simulink model "main"  (R2022a)
settings: Solver=FixedStepDiscrete  StartTime=0.0  StopTime=Inf  FixedStep=(50e-6)-(sim_en*4.995e-5)  RelTol=1e-3  EnableMultiTasking=on
model workspace (MAT data in the model file):
  Param = Simulink.Parameter
  Param.DataType = 'auto'
  Param.Complexity = 'real'
  Param.Dimensions = [0 0]
  ac_ok = Simulink.Signal
  ac_ok.DataType = 'boolean'
  ac_ok.Dimensions = -1
  ac_ok.DimensionsMode = 'Fixed'
  ac_ok.Complexity = 'real'
  ac_ok.SampleTime = -1
  ac_ok.SamplingMode = 'auto'
  ac_ok.InitialValue = '0'
  ac_ok_120 = Simulink.Signal
  ac_ok_120.DataType = 'boolean'
  ac_ok_120.Dimensions = -1
  ac_ok_120.DimensionsMode = 'Fixed'
  ac_ok_120.Complexity = 'real'
  ac_ok_120.SampleTime = -1
  ac_ok_120.SamplingMode = 'auto'
  ac_ok_120.InitialValue = '0'
  bulk_voltage = Simulink.Signal
  bulk_voltage.DataType = 'uint16'
  bulk_voltage.Dimensions = -1
  bulk_voltage.DimensionsMode = 'Fixed'
  bulk_voltage.Complexity = 'real'
  bulk_voltage.SampleTime = -1
  bulk_voltage.SamplingMode = 'auto'
  bulk_voltage.InitialValue = '99'
  burstduty_integ_max = Simulink.Signal
  burstduty_integ_max.DataType = 'single'
  burstduty_integ_max.Dimensions = -1
  burstduty_integ_max.DimensionsMode = 'Fixed'
  burstduty_integ_max.Complexity = 'real'
  burstduty_integ_max.SampleTime = -1
  burstduty_integ_max.SamplingMode = 'auto'
  burstduty_integ_max.InitialValue = '1'
  burstduty_integ_min = Simulink.Signal
  burstduty_integ_min.DataType = 'single'
  burstduty_integ_min.Dimensions = -1
  burstduty_integ_min.DimensionsMode = 'Fixed'
  burstduty_integ_min.Complexity = 'real'
  burstduty_integ_min.SampleTime = -1
  burstduty_integ_min.SamplingMode = 'auto'
  burstduty_integ_min.InitialValue = '1'
  burstduty_ki = Simulink.Signal
  burstduty_ki.DataType = 'single'
  burstduty_ki.Dimensions = -1
  burstduty_ki.DimensionsMode = 'Fixed'
  burstduty_ki.Complexity = 'real'
  burstduty_ki.SampleTime = -1
  burstduty_ki.SamplingMode = 'auto'
  burstduty_ki.InitialValue = '-1'
  burstduty_kp = Simulink.Signal
  burstduty_kp.DataType = 'single'
  burstduty_kp.Dimensions = -1
  burstduty_kp.DimensionsMode = 'Fixed'
  burstduty_kp.Complexity = 'real'
  burstduty_kp.SampleTime = -1
  burstduty_kp.SamplingMode = 'auto'
  burstduty_kp.InitialValue = '-1'
  calib_ok = Simulink.Signal
  calib_ok.DataType = 'boolean'
  calib_ok.Dimensions = -1
  calib_ok.DimensionsMode = 'Fixed'
  calib_ok.Complexity = 'real'
  calib_ok.SampleTime = -1
  calib_ok.SamplingMode = 'auto'
  calib_ok.InitialValue = '0'
  can_addr1 = Simulink.Signal
  can_addr1.DataType = 'boolean'
  can_addr1.Dimensions = -1
  can_addr1.DimensionsMode = 'Fixed'
  can_addr1.Complexity = 'real'
  can_addr1.SampleTime = -1
  can_addr1.SamplingMode = 'auto'
  can_addr1.InitialValue = '0'
  can_addr2 = Simulink.Signal
  can_addr2.DataType = 'boolean'
  can_addr2.Dimensions = -1
  can_addr2.DimensionsMode = 'Fixed'
  can_addr2.Complexity = 'real'
  can_addr2.SampleTime = -1
  can_addr2.SamplingMode = 'auto'
  can_addr2.InitialValue = '0'
  can_addr3 = Simulink.Signal
  can_addr3.DataType = 'boolean'
  can_addr3.Dimensions = -1
  can_addr3.DimensionsMode = 'Fixed'
  can_addr3.Complexity = 'real'
  can_addr3.SampleTime = -1
  can_addr3.SamplingMode = 'auto'
  can_addr3.InitialValue = '0'
  can_addr4 = Simulink.Signal
  can_addr4.DataType = 'boolean'
  can_addr4.Dimensions = -1
  can_addr4.DimensionsMode = 'Fixed'
  can_addr4.Complexity = 'real'
  can_addr4.SampleTime = -1
  can_addr4.SamplingMode = 'auto'
  can_addr4.InitialValue = '0'
  can_data_rx = Simulink.Signal
  can_data_rx.DataType = 'uint8'
  can_data_rx.Dimensions = [1 8]
  can_data_rx.DimensionsMode = 'Fixed'
  can_data_rx.Complexity = 'real'
  can_data_rx.SampleTime = -1
  can_data_rx.SamplingMode = 'auto'
  can_data_rx.InitialValue = '[0 0 0 0 0 0 0 0]'
  can_data_tx = Simulink.Signal
  can_data_tx.DataType = 'uint8'
  can_data_tx.Dimensions = [1 8]
  can_data_tx.DimensionsMode = 'Fixed'
  can_data_tx.Complexity = 'real'
  can_data_tx.SampleTime = -1
  can_data_tx.SamplingMode = 'auto'
  can_data_tx.InitialValue = '[0 0 0 0 0 0 0 0]'
  can_timeout_120 = Simulink.Signal
  can_timeout_120.DataType = 'boolean'
  can_timeout_120.Dimensions = -1
  can_timeout_120.DimensionsMode = 'Fixed'
  can_timeout_120.Complexity = 'real'
  can_timeout_120.SampleTime = -1
  can_timeout_120.SamplingMode = 'auto'
  can_timeout_120.InitialValue = '0'
  chksum_scircv = Simulink.Signal
  chksum_scircv.DataType = 'boolean'
  chksum_scircv.Dimensions = -1
  chksum_scircv.DimensionsMode = 'Fixed'
  chksum_scircv.Complexity = 'real'
  chksum_scircv.SampleTime = -1
  chksum_scircv.SamplingMode = 'auto'
  chksum_scircv.InitialValue = '0'
  clllc_en_120 = Simulink.Signal
  clllc_en_120.DataType = 'boolean'
  clllc_en_120.Dimensions = -1
  clllc_en_120.DimensionsMode = 'Fixed'
  clllc_en_120.Complexity = 'real'
  clllc_en_120.SampleTime = -1
  clllc_en_120.SamplingMode = 'auto'
  clllc_en_120.InitialValue = '0'
  clllc_fault_120 = Simulink.Signal
  clllc_fault_120.DataType = 'boolean'
  clllc_fault_120.Dimensions = -1
  clllc_fault_120.DimensionsMode = 'Fixed'
  clllc_fault_120.Complexity = 'real'
  clllc_fault_120.SampleTime = -1
  clllc_fault_120.SamplingMode = 'auto'
  clllc_fault_120.InitialValue = '0'
  clllc_ok_120 = Simulink.Signal
  clllc_ok_120.DataType = 'boolean'
  clllc_ok_120.Dimensions = -1
  clllc_ok_120.DimensionsMode = 'Fixed'
  clllc_ok_120.Complexity = 'real'
  clllc_ok_120.SampleTime = -1
  clllc_ok_120.SamplingMode = 'auto'
  clllc_ok_120.InitialValue = '0'
  cmpss1h = Simulink.Signal
  cmpss1h.DataType = 'boolean'
  cmpss1h.Dimensions = -1
  cmpss1h.DimensionsMode = 'Fixed'
  cmpss1h.Complexity = 'real'
  cmpss1h.SampleTime = -1
  cmpss1h.SamplingMode = 'auto'
  cmpss1h.InitialValue = '0'
  cmpss1l = Simulink.Signal
  cmpss1l.DataType = 'boolean'
  cmpss1l.Dimensions = -1
  cmpss1l.DimensionsMode = 'Fixed'
  cmpss1l.Complexity = 'real'
  cmpss1l.SampleTime = -1
  cmpss1l.SamplingMode = 'auto'
  cmpss1l.InitialValue = '0'
  cmpss2h = Simulink.Signal
  cmpss2h.DataType = 'boolean'
  cmpss2h.Dimensions = -1
  cmpss2h.DimensionsMode = 'Fixed'
  cmpss2h.Complexity = 'real'
  cmpss2h.SampleTime = -1
  cmpss2h.SamplingMode = 'auto'
  cmpss2h.InitialValue = '0'
  cmpss2l = Simulink.Signal
  cmpss2l.DataType = 'boolean'
  cmpss2l.Dimensions = -1
  cmpss2l.DimensionsMode = 'Fixed'
  cmpss2l.Complexity = 'real'
  cmpss2l.SampleTime = -1
  cmpss2l.SamplingMode = 'auto'
  cmpss2l.InitialValue = '0'
  cmpss3h = Simulink.Signal
  cmpss3h.DataType = 'boolean'
  cmpss3h.Dimensions = -1
  cmpss3h.DimensionsMode = 'Fixed'
  cmpss3h.Complexity = 'real'
  cmpss3h.SampleTime = -1
  cmpss3h.SamplingMode = 'auto'
  cmpss3h.InitialValue = '0'
  cmpss3l = Simulink.Signal
  cmpss3l.DataType = 'boolean'
  cmpss3l.Dimensions = -1
  cmpss3l.DimensionsMode = 'Fixed'
  cmpss3l.Complexity = 'real'
  cmpss3l.SampleTime = -1
  cmpss3l.SamplingMode = 'auto'
  cmpss3l.InitialValue = '0'
  cmpss4h = Simulink.Signal
  cmpss4h.DataType = 'boolean'
  cmpss4h.Dimensions = -1
  cmpss4h.DimensionsMode = 'Fixed'
  cmpss4h.Complexity = 'real'
  cmpss4h.SampleTime = -1
  cmpss4h.SamplingMode = 'auto'
  cmpss4h.InitialValue = '0'
  cmpss4l = Simulink.Signal
  cmpss4l.DataType = 'boolean'
  cmpss4l.Dimensions = -1
  cmpss4l.DimensionsMode = 'Fixed'
  cmpss4l.Complexity = 'real'
  cmpss4l.SampleTime = -1
  cmpss4l.SamplingMode = 'auto'
  cmpss4l.InitialValue = '0'
  cmpss5h = Simulink.Signal
  cmpss5h.DataType = 'boolean'
  cmpss5h.Dimensions = -1
  cmpss5h.DimensionsMode = 'Fixed'
  cmpss5h.Complexity = 'real'
  cmpss5h.SampleTime = -1
  cmpss5h.SamplingMode = 'auto'
  cmpss5h.InitialValue = '0'
  cmpss5l = Simulink.Signal
  cmpss5l.DataType = 'boolean'
  cmpss5l.Dimensions = -1
  cmpss5l.DimensionsMode = 'Fixed'
  cmpss5l.Complexity = 'real'
  cmpss5l.SampleTime = -1
  cmpss5l.SamplingMode = 'auto'
  cmpss5l.InitialValue = '0'
  cmpss6h = Simulink.Signal
  cmpss6h.DataType = 'boolean'
  cmpss6h.Dimensions = -1
  cmpss6h.DimensionsMode = 'Fixed'
  cmpss6h.Complexity = 'real'
  cmpss6h.SampleTime = -1
  cmpss6h.SamplingMode = 'auto'
  cmpss6h.InitialValue = '0'
  cmpss6l = Simulink.Signal
  cmpss6l.DataType = 'boolean'
  cmpss6l.Dimensions = -1
  cmpss6l.DimensionsMode = 'Fixed'
  cmpss6l.Complexity = 'real'
  cmpss6l.SampleTime = -1
  cmpss6l.SamplingMode = 'auto'
  cmpss6l.InitialValue = '0'
  cmpss7h = Simulink.Signal
  cmpss7h.DataType = 'boolean'
  cmpss7h.Dimensions = -1
  cmpss7h.DimensionsMode = 'Fixed'
  cmpss7h.Complexity = 'real'
  cmpss7h.SampleTime = -1
  cmpss7h.SamplingMode = 'auto'
  cmpss7h.InitialValue = '0'
  cmpss7l = Simulink.Signal
  cmpss7l.DataType = 'boolean'
  cmpss7l.Dimensions = -1
  cmpss7l.DimensionsMode = 'Fixed'
  cmpss7l.Complexity = 'real'
  cmpss7l.SampleTime = -1
  cmpss7l.SamplingMode = 'auto'
  cmpss7l.InitialValue = '0'
  cmpss8h = Simulink.Signal
  cmpss8h.DataType = 'boolean'
  cmpss8h.Dimensions = -1
  cmpss8h.DimensionsMode = 'Fixed'
  cmpss8h.Complexity = 'real'
  cmpss8h.SampleTime = -1
  cmpss8h.SamplingMode = 'auto'
  cmpss8h.InitialValue = '0'
  cmpss8l = Simulink.Signal
  cmpss8l.DataType = 'boolean'
  cmpss8l.Dimensions = -1
  cmpss8l.DimensionsMode = 'Fixed'
  cmpss8l.Complexity = 'real'
  cmpss8l.SampleTime = -1
  cmpss8l.SamplingMode = 'auto'
  cmpss8l.InitialValue = '0'
  cnt_idle = Simulink.Signal
  cnt_idle.DataType = 'uint16'
  cnt_idle.Dimensions = -1
  cnt_idle.DimensionsMode = 'Fixed'
  cnt_idle.Complexity = 'real'
  cnt_idle.SampleTime = -1
  cnt_idle.SamplingMode = 'auto'
  cnt_idle.InitialValue = '0'
  cnt_orps = Simulink.Signal
  cnt_orps.DataType = 'uint16'
  cnt_orps.Dimensions = -1
  cnt_orps.DimensionsMode = 'Fixed'
  cnt_orps.Complexity = 'real'
  cnt_orps.SampleTime = -1
  cnt_orps.SamplingMode = 'auto'
  cnt_orps.InitialValue = '0'
  cnt_scircv = Simulink.Signal
  cnt_scircv.DataType = 'uint8'
  cnt_scircv.Dimensions = -1
  cnt_scircv.DimensionsMode = 'Fixed'
  cnt_scircv.Complexity = 'real'
  cnt_scircv.SampleTime = -1
  cnt_scircv.SamplingMode = 'auto'
  cnt_scircv.InitialValue = '0'
  cnt_scixmt = Simulink.Signal
  cnt_scixmt.DataType = 'uint8'
  cnt_scixmt.Dimensions = -1
  cnt_scixmt.DimensionsMode = 'Fixed'
  cnt_scixmt.Complexity = 'real'
  cnt_scixmt.SampleTime = -1
  cnt_scixmt.SamplingMode = 'auto'
  cnt_scixmt.InitialValue = '0'
  cnt_scixmt_func = Simulink.Signal
  cnt_scixmt_func.DataType = 'uint8'
  cnt_scixmt_func.Dimensions = -1
  cnt_scixmt_func.DimensionsMode = 'Fixed'
  cnt_scixmt_func.Complexity = 'real'
  cnt_scixmt_func.SampleTime = -1
  cnt_scixmt_func.SamplingMode = 'auto'
  cnt_scixmt_func.InitialValue = '0'
  cnt_temp_mux = Simulink.Signal
  cnt_temp_mux.DataType = 'uint16'
  cnt_temp_mux.Dimensions = -1
  cnt_temp_mux.DimensionsMode = 'Fixed'
  cnt_temp_mux.Complexity = 'real'
  cnt_temp_mux.SampleTime = -1
  cnt_temp_mux.SamplingMode = 'auto'
  cnt_temp_mux.InitialValue = '0'
  cnt_vdroop = Simulink.Signal
  cnt_vdroop.DataType = 'uint16'
  cnt_vdroop.Dimensions = -1
  cnt_vdroop.DimensionsMode = 'Fixed'
  cnt_vdroop.Complexity = 'real'
  cnt_vdroop.SampleTime = -1
  cnt_vdroop.SamplingMode = 'auto'
  cnt_vdroop.InitialValue = '0'
  config_ok = Simulink.Signal
  config_ok.DataType = 'boolean'
  config_ok.Dimensions = -1
  config_ok.DimensionsMode = 'Fixed'
  config_ok.Complexity = 'real'
  config_ok.SampleTime = -1
  config_ok.SamplingMode = 'auto'
  config_ok.InitialValue = '0'
  control_en = Simulink.Signal
  control_en.DataType = 'boolean'
  control_en.Dimensions = -1
  control_en.DimensionsMode = 'Fixed'
  control_en.Complexity = 'real'
  control_en.SampleTime = -1
  control_en.SamplingMode = 'auto'
  control_en.InitialValue = '0'
  cp_ready_120 = Simulink.Signal
  cp_ready_120.DataType = 'boolean'
  cp_ready_120.Dimensions = -1
  cp_ready_120.DimensionsMode = 'Fixed'
  cp_ready_120.Complexity = 'real'
  cp_ready_120.SampleTime = -1
  cp_ready_120.SamplingMode = 'auto'
  cp_ready_120.InitialValue = '0'
  d2d_en = Simulink.Signal
  d2d_en.DataType = 'boolean'
  d2d_en.Dimensions = -1
  d2d_en.DimensionsMode = 'Fixed'
  d2d_en.Complexity = 'real'
  d2d_en.SampleTime = -1
  d2d_en.SamplingMode = 'auto'
  d2d_en.InitialValue = '1'
  dchg_off = Simulink.Signal
  dchg_off.DataType = 'boolean'
  dchg_off.Dimensions = -1
  dchg_off.DimensionsMode = 'Fixed'
  dchg_off.Complexity = 'real'
  dchg_off.SampleTime = -1
  dchg_off.SamplingMode = 'auto'
  dchg_off.InitialValue = '1'
  debug_dacb = Simulink.Signal
  debug_dacb.DataType = 'uint16'
  debug_dacb.Dimensions = -1
  debug_dacb.DimensionsMode = 'Fixed'
  debug_dacb.Complexity = 'real'
  debug_dacb.SampleTime = -1
  debug_dacb.SamplingMode = 'auto'
  debug_dacb.InitialValue = '0'
  debug_dacc = Simulink.Signal
  debug_dacc.DataType = 'uint16'
  debug_dacc.Dimensions = -1
  debug_dacc.DimensionsMode = 'Fixed'
  debug_dacc.Complexity = 'real'
  debug_dacc.SampleTime = -1
  debug_dacc.SamplingMode = 'auto'
  debug_dacc.InitialValue = '0'
  debug_msg1 = Simulink.Signal
  debug_msg1.DataType = 'uint16'
  debug_msg1.Dimensions = -1
  debug_msg1.DimensionsMode = 'Fixed'
  debug_msg1.Complexity = 'real'
  debug_msg1.SampleTime = -1
  debug_msg1.SamplingMode = 'auto'
  debug_msg1.InitialValue = '99'
  debug_msg2 = Simulink.Signal
  debug_msg2.DataType = 'uint16'
  debug_msg2.Dimensions = -1
  debug_msg2.DimensionsMode = 'Fixed'
  debug_msg2.Complexity = 'real'
  debug_msg2.SampleTime = -1
  debug_msg2.SamplingMode = 'auto'
  debug_msg2.InitialValue = '99'
  debug_msg3 = Simulink.Signal
  debug_msg3.DataType = 'uint16'
  debug_msg3.Dimensions = -1
  debug_msg3.DimensionsMode = 'Fixed'
  debug_msg3.Complexity = 'real'
  debug_msg3.SampleTime = -1
  debug_msg3.SamplingMode = 'auto'
  debug_msg3.InitialValue = '99'
  debug_msg4 = Simulink.Signal
  debug_msg4.DataType = 'uint16'
  debug_msg4.Dimensions = -1
  debug_msg4.DimensionsMode = 'Fixed'
  debug_msg4.Complexity = 'real'
  debug_msg4.SampleTime = -1
  debug_msg4.SamplingMode = 'auto'
  debug_msg4.InitialValue = '99'
  debug_msg5 = Simulink.Signal
  debug_msg5.DataType = 'uint16'
  debug_msg5.Dimensions = -1
  debug_msg5.DimensionsMode = 'Fixed'
  debug_msg5.Complexity = 'real'
  debug_msg5.SampleTime = -1
  debug_msg5.SamplingMode = 'auto'
  debug_msg5.InitialValue = '99'
  debug_msg6 = Simulink.Signal
  debug_msg6.DataType = 'uint16'
  debug_msg6.Dimensions = -1
  debug_msg6.DimensionsMode = 'Fixed'
  debug_msg6.Complexity = 'real'
  debug_msg6.SampleTime = -1
  debug_msg6.SamplingMode = 'auto'
  debug_msg6.InitialValue = '99'
  dir_v2g = Simulink.Signal
  dir_v2g.DataType = 'boolean'
  dir_v2g.Dimensions = -1
  dir_v2g.DimensionsMode = 'Fixed'
  dir_v2g.Complexity = 'real'
  dir_v2g.SampleTime = -1
  dir_v2g.SamplingMode = 'auto'
  dir_v2g.InitialValue = '0'
  eoss_llc1 = Simulink.Signal
  eoss_llc1.DataType = 'boolean'
  eoss_llc1.Dimensions = -1
  eoss_llc1.DimensionsMode = 'Fixed'
  eoss_llc1.Complexity = 'real'
  eoss_llc1.SampleTime = -1
  eoss_llc1.SamplingMode = 'auto'
  eoss_llc1.InitialValue = '0'
  eoss_llc2 = Simulink.Signal
  eoss_llc2.DataType = 'boolean'
  eoss_llc2.Dimensions = -1
  eoss_llc2.DimensionsMode = 'Fixed'
  eoss_llc2.Complexity = 'real'
  eoss_llc2.SampleTime = -1
  eoss_llc2.SamplingMode = 'auto'
  eoss_llc2.InitialValue = '0'
  eoss_orps = Simulink.Signal
  eoss_orps.DataType = 'boolean'
  eoss_orps.Dimensions = -1
  eoss_orps.DimensionsMode = 'Fixed'
  eoss_orps.Complexity = 'real'
  eoss_orps.SampleTime = -1
  eoss_orps.SamplingMode = 'auto'
  eoss_orps.InitialValue = '0'
  fault_ocp = Simulink.Signal
  fault_ocp.DataType = 'boolean'
  fault_ocp.Dimensions = -1
  fault_ocp.DimensionsMode = 'Fixed'
  fault_ocp.Complexity = 'real'
  fault_ocp.SampleTime = -1
  fault_ocp.SamplingMode = 'auto'
  fault_ocp.InitialValue = '0'
  fault_otp = Simulink.Signal
  fault_otp.DataType = 'boolean'
  fault_otp.Dimensions = -1
  fault_otp.DimensionsMode = 'Fixed'
  fault_otp.Complexity = 'real'
  fault_otp.SampleTime = -1
  fault_otp.SamplingMode = 'auto'
  fault_otp.InitialValue = '0'
  fault_ovp = Simulink.Signal
  fault_ovp.DataType = 'boolean'
  fault_ovp.Dimensions = -1
  fault_ovp.DimensionsMode = 'Fixed'
  fault_ovp.Complexity = 'real'
  fault_ovp.SampleTime = -1
  fault_ovp.SamplingMode = 'auto'
  fault_ovp.InitialValue = '0'
  fut_en = Simulink.Signal
  fut_en.DataType = 'boolean'
  fut_en.Dimensions = -1
  fut_en.DimensionsMode = 'Fixed'
  fut_en.Complexity = 'real'
  fut_en.SampleTime = -1
  fut_en.SamplingMode = 'auto'
  fut_en.InitialValue = '0'
  fwd_en_120 = Simulink.Signal
  fwd_en_120.DataType = 'boolean'
  fwd_en_120.Dimensions = -1
  fwd_en_120.DimensionsMode = 'Fixed'
  fwd_en_120.Complexity = 'real'
  fwd_en_120.SampleTime = -1
  fwd_en_120.SamplingMode = 'auto'
  fwd_en_120.InitialValue = '0'
  gain_llc1_sec_idc = Simulink.Signal
  gain_llc1_sec_idc.DataType = 'single'
  gain_llc1_sec_idc.Dimensions = -1
  gain_llc1_sec_idc.DimensionsMode = 'Fixed'
  gain_llc1_sec_idc.Complexity = 'real'
  gain_llc1_sec_idc.SampleTime = -1
  gain_llc1_sec_idc.SamplingMode = 'auto'
  gain_llc1_sec_idc.InitialValue = '(4095/3.3)*(0.02)'
  gain_llc1_temp_sr = Simulink.Signal
  gain_llc1_temp_sr.DataType = 'single'
  gain_llc1_temp_sr.Dimensions = -1
  gain_llc1_temp_sr.DimensionsMode = 'Fixed'
  gain_llc1_temp_sr.Complexity = 'real'
  gain_llc1_temp_sr.SampleTime = -1
  gain_llc1_temp_sr.SamplingMode = 'auto'
  gain_llc1_temp_sr.InitialValue = '1'
  gain_llc2_sec_idc = Simulink.Signal
  gain_llc2_sec_idc.DataType = 'single'
  gain_llc2_sec_idc.Dimensions = -1
  gain_llc2_sec_idc.DimensionsMode = 'Fixed'
  gain_llc2_sec_idc.Complexity = 'real'
  gain_llc2_sec_idc.SampleTime = -1
  gain_llc2_sec_idc.SamplingMode = 'auto'
  gain_llc2_sec_idc.InitialValue = '24.8188'
  gain_vbat = Simulink.Signal
  gain_vbat.DataType = 'single'
  gain_vbat.Dimensions = -1
  gain_vbat.DimensionsMode = 'Fixed'
  gain_vbat.Complexity = 'real'
  gain_vbat.SampleTime = -1
  gain_vbat.SamplingMode = 'auto'
  gain_vbat.InitialValue = '(4095/3.3)*(0.00569)'
  gain_vbulk = Simulink.Signal
  gain_vbulk.DataType = 'single'
  gain_vbulk.Dimensions = -1
  gain_vbulk.DimensionsMode = 'Fixed'
  gain_vbulk.Complexity = 'real'
  gain_vbulk.SampleTime = -1
  gain_vbulk.SamplingMode = 'auto'
  gain_vbulk.InitialValue = '(4095/3.3)*(0.00272)'
  gain_vout = Simulink.Signal
  gain_vout.DataType = 'single'
  gain_vout.Dimensions = -1
  gain_vout.DimensionsMode = 'Fixed'
  gain_vout.Complexity = 'real'
  gain_vout.SampleTime = -1
  gain_vout.SamplingMode = 'auto'
  gain_vout.InitialValue = '(4095/3.3)*(0.00569)'
  input_current_phasea = Simulink.Signal
  input_current_phasea.DataType = 'uint16'
  input_current_phasea.Dimensions = -1
  input_current_phasea.DimensionsMode = 'Fixed'
  input_current_phasea.Complexity = 'real'
  input_current_phasea.SampleTime = -1
  input_current_phasea.SamplingMode = 'auto'
  input_current_phasea.InitialValue = '99'
  input_current_phaseb = Simulink.Signal
  input_current_phaseb.DataType = 'uint16'
  input_current_phaseb.Dimensions = -1
  input_current_phaseb.DimensionsMode = 'Fixed'
  input_current_phaseb.Complexity = 'real'
  input_current_phaseb.SampleTime = -1
  input_current_phaseb.SamplingMode = 'auto'
  input_current_phaseb.InitialValue = '99'
  input_current_phasec = Simulink.Signal
  input_current_phasec.DataType = 'uint16'
  input_current_phasec.Dimensions = -1
  input_current_phasec.DimensionsMode = 'Fixed'
  input_current_phasec.Complexity = 'real'
  input_current_phasec.SampleTime = -1
  input_current_phasec.SamplingMode = 'auto'
  input_current_phasec.InitialValue = '99'
  input_freq = Simulink.Signal
  input_freq.DataType = 'uint16'
  input_freq.Dimensions = -1
  input_freq.DimensionsMode = 'Fixed'
  input_freq.Complexity = 'real'
  input_freq.SampleTime = -1
  input_freq.SamplingMode = 'auto'
  input_freq.InitialValue = '99'
  input_power = Simulink.Signal
  input_power.DataType = 'uint16'
  input_power.Dimensions = -1
  input_power.DimensionsMode = 'Fixed'
  input_power.Complexity = 'real'
  input_power.SampleTime = -1
  input_power.SamplingMode = 'auto'
  input_power.InitialValue = '99'
  input_voltage_phasea = Simulink.Signal
  input_voltage_phasea.DataType = 'uint16'
  input_voltage_phasea.Dimensions = -1
  input_voltage_phasea.DimensionsMode = 'Fixed'
  input_voltage_phasea.Complexity = 'real'
  input_voltage_phasea.SampleTime = -1
  input_voltage_phasea.SamplingMode = 'auto'
  input_voltage_phasea.InitialValue = '99'
  input_voltage_phaseb = Simulink.Signal
  input_voltage_phaseb.DataType = 'uint16'
  input_voltage_phaseb.Dimensions = -1
  input_voltage_phaseb.DimensionsMode = 'Fixed'
  input_voltage_phaseb.Complexity = 'real'
  input_voltage_phaseb.SampleTime = -1
  input_voltage_phaseb.SamplingMode = 'auto'
  input_voltage_phaseb.InitialValue = '99'
  input_voltage_phasec = Simulink.Signal
  input_voltage_phasec.DataType = 'uint16'
  input_voltage_phasec.Dimensions = -1
  input_voltage_phasec.DimensionsMode = 'Fixed'
  input_voltage_phasec.Complexity = 'real'
  input_voltage_phasec.SampleTime = -1
  input_voltage_phasec.SamplingMode = 'auto'
  input_voltage_phasec.InitialValue = '99'
  ishare_arbiter = Simulink.Signal
  ishare_arbiter.DataType = 'uint16'
  ishare_arbiter.Dimensions = -1
  ishare_arbiter.DimensionsMode = 'Fixed'
  ishare_arbiter.Complexity = 'real'
  ishare_arbiter.SampleTime = -1
  ishare_arbiter.SamplingMode = 'auto'
  ishare_arbiter.InitialValue = '37'
  ishare_thresh = Simulink.Signal
  ishare_thresh.DataType = 'uint16'
  ishare_thresh.Dimensions = -1
  ishare_thresh.DimensionsMode = 'Fixed'
  ishare_thresh.Complexity = 'real'
  ishare_thresh.SampleTime = -1
  ishare_thresh.SamplingMode = 'auto'
  ishare_thresh.InitialValue = '372'
  led_g = Simulink.Signal
  led_g.DataType = 'boolean'
  led_g.Dimensions = -1
  led_g.DimensionsMode = 'Fixed'
  led_g.Complexity = 'real'
  led_g.SampleTime = -1
  led_g.SamplingMode = 'auto'
  led_g.InitialValue = '0'
  led_r = Simulink.Signal
  led_r.DataType = 'boolean'
  led_r.Dimensions = -1
  led_r.DimensionsMode = 'Fixed'
  led_r.Complexity = 'real'
  led_r.SampleTime = -1
  led_r.SamplingMode = 'auto'
  led_r.InitialValue = '0'
  led_y = Simulink.Signal
  led_y.DataType = 'boolean'
  led_y.Dimensions = -1
  led_y.DimensionsMode = 'Fixed'
  led_y.Complexity = 'real'
  led_y.SampleTime = -1
  led_y.SamplingMode = 'auto'
  led_y.InitialValue = '0'
  llc1_burst_integ = Simulink.Signal
  llc1_burst_integ.DataType = 'single'
  llc1_burst_integ.Dimensions = -1
  llc1_burst_integ.DimensionsMode = 'Fixed'
  llc1_burst_integ.Complexity = 'real'
  llc1_burst_integ.SampleTime = -1
  llc1_burst_integ.SamplingMode = 'auto'
  llc1_burst_integ.InitialValue = '0'
  llc1_burstduty_buffer = Simulink.Signal
  llc1_burstduty_buffer.DataType = 'single'
  llc1_burstduty_buffer.Dimensions = -1
  llc1_burstduty_buffer.DimensionsMode = 'Fixed'
  llc1_burstduty_buffer.Complexity = 'real'
  llc1_burstduty_buffer.SampleTime = -1
  llc1_burstduty_buffer.SamplingMode = 'auto'
  llc1_burstduty_buffer.InitialValue = '100'
  llc1_pfm_error = Simulink.Signal
  llc1_pfm_error.DataType = 'uint16'
  llc1_pfm_error.Dimensions = -1
  llc1_pfm_error.DimensionsMode = 'Fixed'
  llc1_pfm_error.Complexity = 'real'
  llc1_pfm_error.SampleTime = -1
  llc1_pfm_error.SamplingMode = 'auto'
  llc1_pfm_error.InitialValue = '0'
  llc1_pfm_integ = Simulink.Signal
  llc1_pfm_integ.DataType = 'single'
  llc1_pfm_integ.Dimensions = -1
  llc1_pfm_integ.DimensionsMode = 'Fixed'
  llc1_pfm_integ.Complexity = 'real'
  llc1_pfm_integ.SampleTime = -1
  llc1_pfm_integ.SamplingMode = 'auto'
  llc1_pfm_integ.InitialValue = '0'
  llc1_pfm_prop = Simulink.Signal
  llc1_pfm_prop.DataType = 'uint16'
  llc1_pfm_prop.Dimensions = -1
  llc1_pfm_prop.DimensionsMode = 'Fixed'
  llc1_pfm_prop.Complexity = 'real'
  llc1_pfm_prop.SampleTime = -1
  llc1_pfm_prop.SamplingMode = 'auto'
  llc1_pfm_prop.InitialValue = '0'
  llc1_pri_idc = Simulink.Signal
  llc1_pri_idc.DataType = 'single'
  llc1_pri_idc.Dimensions = -1
  llc1_pri_idc.DimensionsMode = 'Fixed'
  llc1_pri_idc.Complexity = 'real'
  llc1_pri_idc.SampleTime = -1
  llc1_pri_idc.SamplingMode = 'auto'
  llc1_pri_idc.InitialValue = '0'
  llc1_ps_buffer = Simulink.Signal
  llc1_ps_buffer.DataType = 'single'
  llc1_ps_buffer.Dimensions = -1
  llc1_ps_buffer.DimensionsMode = 'Fixed'
  llc1_ps_buffer.Complexity = 'real'
  llc1_ps_buffer.SampleTime = -1
  llc1_ps_buffer.SamplingMode = 'auto'
  llc1_ps_buffer.InitialValue = '45'
  llc1_pspwm_error = Simulink.Signal
  llc1_pspwm_error.DataType = 'uint16'
  llc1_pspwm_error.Dimensions = -1
  llc1_pspwm_error.DimensionsMode = 'Fixed'
  llc1_pspwm_error.Complexity = 'real'
  llc1_pspwm_error.SampleTime = -1
  llc1_pspwm_error.SamplingMode = 'auto'
  llc1_pspwm_error.InitialValue = '0'
  llc1_pspwm_integ = Simulink.Signal
  llc1_pspwm_integ.DataType = 'single'
  llc1_pspwm_integ.Dimensions = -1
  llc1_pspwm_integ.DimensionsMode = 'Fixed'
  llc1_pspwm_integ.Complexity = 'real'
  llc1_pspwm_integ.SampleTime = -1
  llc1_pspwm_integ.SamplingMode = 'auto'
  llc1_pspwm_integ.InitialValue = '0'
  llc1_pspwm_prop = Simulink.Signal
  llc1_pspwm_prop.DataType = 'uint16'
  llc1_pspwm_prop.Dimensions = -1
  llc1_pspwm_prop.DimensionsMode = 'Fixed'
  llc1_pspwm_prop.Complexity = 'real'
  llc1_pspwm_prop.SampleTime = -1
  llc1_pspwm_prop.SamplingMode = 'auto'
  llc1_pspwm_prop.InitialValue = '0'
  llc1_sec_idc = Simulink.Signal
  llc1_sec_idc.DataType = 'single'
  llc1_sec_idc.Dimensions = -1
  llc1_sec_idc.DimensionsMode = 'Fixed'
  llc1_sec_idc.Complexity = 'real'
  llc1_sec_idc.SampleTime = -1
  llc1_sec_idc.SamplingMode = 'auto'
  llc1_sec_idc.InitialValue = '1'
  llc1_temp_sr = Simulink.Signal
  llc1_temp_sr.DataType = 'uint16'
  llc1_temp_sr.Dimensions = -1
  llc1_temp_sr.DimensionsMode = 'Fixed'
  llc1_temp_sr.Complexity = 'real'
  llc1_temp_sr.SampleTime = -1
  llc1_temp_sr.SamplingMode = 'auto'
  llc1_temp_sr.InitialValue = '1'
  llc1_ts_tbctr_buffer = Simulink.Signal
  llc1_ts_tbctr_buffer.DataType = 'single'
  llc1_ts_tbctr_buffer.Dimensions = -1
  llc1_ts_tbctr_buffer.DimensionsMode = 'Fixed'
  llc1_ts_tbctr_buffer.Complexity = 'real'
  llc1_ts_tbctr_buffer.SampleTime = -1
  llc1_ts_tbctr_buffer.SamplingMode = 'auto'
  llc1_ts_tbctr_buffer.InitialValue = '100'
  llc2_burst_integ = Simulink.Signal
  llc2_burst_integ.DataType = 'single'
  llc2_burst_integ.Dimensions = -1
  llc2_burst_integ.DimensionsMode = 'Fixed'
  llc2_burst_integ.Complexity = 'real'
  llc2_burst_integ.SampleTime = -1
  llc2_burst_integ.SamplingMode = 'auto'
  llc2_burst_integ.InitialValue = '0'
  llc2_burstduty_buffer = Simulink.Signal
  llc2_burstduty_buffer.DataType = 'single'
  llc2_burstduty_buffer.Dimensions = -1
  llc2_burstduty_buffer.DimensionsMode = 'Fixed'
  llc2_burstduty_buffer.Complexity = 'real'
  llc2_burstduty_buffer.SampleTime = -1
  llc2_burstduty_buffer.SamplingMode = 'auto'
  llc2_burstduty_buffer.InitialValue = '100'
  llc2_en = Simulink.Signal
  llc2_en.DataType = 'boolean'
  llc2_en.Dimensions = -1
  llc2_en.DimensionsMode = 'Fixed'
  llc2_en.Complexity = 'real'
  llc2_en.SampleTime = -1
  llc2_en.SamplingMode = 'auto'
  llc2_en.InitialValue = '0'
  llc2_en_buffer = Simulink.Signal
  llc2_en_buffer.DataType = 'boolean'
  llc2_en_buffer.Dimensions = -1
  llc2_en_buffer.DimensionsMode = 'Fixed'
  llc2_en_buffer.Complexity = 'real'
  llc2_en_buffer.SampleTime = -1
  llc2_en_buffer.SamplingMode = 'auto'
  llc2_en_buffer.InitialValue = '0'
  llc2_pfm_error = Simulink.Signal
  llc2_pfm_error.DataType = 'uint16'
  llc2_pfm_error.Dimensions = -1
  llc2_pfm_error.DimensionsMode = 'Fixed'
  llc2_pfm_error.Complexity = 'real'
  llc2_pfm_error.SampleTime = -1
  llc2_pfm_error.SamplingMode = 'auto'
  llc2_pfm_error.InitialValue = '0'
  llc2_pfm_integ = Simulink.Signal
  llc2_pfm_integ.DataType = 'single'
  llc2_pfm_integ.Dimensions = -1
  llc2_pfm_integ.DimensionsMode = 'Fixed'
  llc2_pfm_integ.Complexity = 'real'
  llc2_pfm_integ.SampleTime = -1
  llc2_pfm_integ.SamplingMode = 'auto'
  llc2_pfm_integ.InitialValue = '0'
  llc2_pfm_prop = Simulink.Signal
  llc2_pfm_prop.DataType = 'uint16'
  llc2_pfm_prop.Dimensions = -1
  llc2_pfm_prop.DimensionsMode = 'Fixed'
  llc2_pfm_prop.Complexity = 'real'
  llc2_pfm_prop.SampleTime = -1
  llc2_pfm_prop.SamplingMode = 'auto'
  llc2_pfm_prop.InitialValue = '0'
  llc2_pri_idc = Simulink.Signal
  llc2_pri_idc.DataType = 'uint16'
  llc2_pri_idc.Dimensions = -1
  llc2_pri_idc.DimensionsMode = 'Fixed'
  llc2_pri_idc.Complexity = 'real'
  llc2_pri_idc.SampleTime = -1
  llc2_pri_idc.SamplingMode = 'auto'
  llc2_pri_idc.InitialValue = '1'
  llc2_ps_buffer = Simulink.Signal
  llc2_ps_buffer.DataType = 'single'
  llc2_ps_buffer.Dimensions = -1
  llc2_ps_buffer.DimensionsMode = 'Fixed'
  llc2_ps_buffer.Complexity = 'real'
  llc2_ps_buffer.SampleTime = -1
  llc2_ps_buffer.SamplingMode = 'auto'
  llc2_ps_buffer.InitialValue = '45'
  llc2_pspwm_error = Simulink.Signal
  llc2_pspwm_error.DataType = 'uint16'
  llc2_pspwm_error.Dimensions = -1
  llc2_pspwm_error.DimensionsMode = 'Fixed'
  llc2_pspwm_error.Complexity = 'real'
  llc2_pspwm_error.SampleTime = -1
  llc2_pspwm_error.SamplingMode = 'auto'
  llc2_pspwm_error.InitialValue = '0'
  llc2_pspwm_integ = Simulink.Signal
  llc2_pspwm_integ.DataType = 'single'
  llc2_pspwm_integ.Dimensions = -1
  llc2_pspwm_integ.DimensionsMode = 'Fixed'
  llc2_pspwm_integ.Complexity = 'real'
  llc2_pspwm_integ.SampleTime = -1
  llc2_pspwm_integ.SamplingMode = 'auto'
  llc2_pspwm_integ.InitialValue = '0'
  llc2_pspwm_prop = Simulink.Signal
  llc2_pspwm_prop.DataType = 'int16'
  llc2_pspwm_prop.Dimensions = -1
  llc2_pspwm_prop.DimensionsMode = 'Fixed'
  llc2_pspwm_prop.Complexity = 'real'
  llc2_pspwm_prop.SampleTime = -1
  llc2_pspwm_prop.SamplingMode = 'auto'
  llc2_pspwm_prop.InitialValue = '0'
  llc2_sec_idc = Simulink.Signal
  llc2_sec_idc.DataType = 'uint16'
  llc2_sec_idc.Dimensions = -1
  llc2_sec_idc.DimensionsMode = 'Fixed'
  llc2_sec_idc.Complexity = 'real'
  llc2_sec_idc.SampleTime = -1
  llc2_sec_idc.SamplingMode = 'auto'
  llc2_sec_idc.InitialValue = '1'
  llc2_temp_sr = Simulink.Signal
  llc2_temp_sr.DataType = 'uint16'
  llc2_temp_sr.Dimensions = -1
  llc2_temp_sr.DimensionsMode = 'Fixed'
  llc2_temp_sr.Complexity = 'real'
  llc2_temp_sr.SampleTime = -1
  llc2_temp_sr.SamplingMode = 'auto'
  llc2_temp_sr.InitialValue = '1'
  llc2_ts_tbctr_buffer = Simulink.Signal
  llc2_ts_tbctr_buffer.DataType = 'single'
  llc2_ts_tbctr_buffer.Dimensions = -1
  llc2_ts_tbctr_buffer.DimensionsMode = 'Fixed'
  llc2_ts_tbctr_buffer.Complexity = 'real'
  llc2_ts_tbctr_buffer.SampleTime = -1
  llc2_ts_tbctr_buffer.SamplingMode = 'auto'
  llc2_ts_tbctr_buffer.InitialValue = '100'
  loop_adcint = Simulink.Signal
  loop_adcint.DataType = 'uint16'
  loop_adcint.Dimensions = -1
  loop_adcint.DimensionsMode = 'Fixed'
  loop_adcint.Complexity = 'real'
  loop_adcint.SampleTime = -1
  loop_adcint.SamplingMode = 'auto'
  loop_adcint.InitialValue = '0'
  loop_control = Simulink.Signal
  loop_control.DataType = 'uint16'
  loop_control.Dimensions = -1
  loop_control.DimensionsMode = 'Fixed'
  loop_control.Complexity = 'real'
  loop_control.SampleTime = -1
  loop_control.SamplingMode = 'auto'
  loop_control.InitialValue = '0'
  loop_idle = Simulink.Signal
  loop_idle.DataType = 'uint16'
  loop_idle.Dimensions = -1
  loop_idle.DimensionsMode = 'Fixed'
  loop_idle.Complexity = 'real'
  loop_idle.SampleTime = -1
  loop_idle.SamplingMode = 'auto'
  loop_idle.InitialValue = '0'
  mid_bulk_voltage = Simulink.Signal
  mid_bulk_voltage.DataType = 'uint16'
  mid_bulk_voltage.Dimensions = -1
  mid_bulk_voltage.DimensionsMode = 'Fixed'
  mid_bulk_voltage.Complexity = 'real'
  mid_bulk_voltage.SampleTime = -1
  mid_bulk_voltage.SamplingMode = 'auto'
  mid_bulk_voltage.InitialValue = '99'
  mode_120 = Simulink.Signal
  mode_120.DataType = 'uint8'
  mode_120.Dimensions = -1
  mode_120.DimensionsMode = 'Fixed'
  mode_120.Complexity = 'real'
  mode_120.SampleTime = -1
  mode_120.SamplingMode = 'auto'
  mode_120.InitialValue = '0'
  mode_cc_cv = Simulink.Signal
  mode_cc_cv.DataType = 'uint8'
  mode_cc_cv.Dimensions = -1
  mode_cc_cv.DimensionsMode = 'Fixed'
  mode_cc_cv.Complexity = 'real'
  mode_cc_cv.SampleTime = -1
  mode_cc_cv.SamplingMode = 'auto'
  mode_cc_cv.InitialValue = '99'
  myParam = mpt.Parameter
  myParam.Value = 1
  myParam.DataType = 'uint16'
  myParam.Complexity = 'real'
  myParam.Dimensions = [1 1]
  obc_ok_120 = Simulink.Signal
  obc_ok_120.DataType = 'boolean'
  obc_ok_120.Dimensions = -1
  obc_ok_120.DimensionsMode = 'Fixed'
  obc_ok_120.Complexity = 'real'
  obc_ok_120.SampleTime = -1
  obc_ok_120.SamplingMode = 'auto'
  obc_ok_120.InitialValue = '0'
  offset_llc1_sec_idc = Simulink.Signal
  offset_llc1_sec_idc.DataType = 'uint16'
  offset_llc1_sec_idc.Dimensions = -1
  offset_llc1_sec_idc.DimensionsMode = 'Fixed'
  offset_llc1_sec_idc.Complexity = 'real'
  offset_llc1_sec_idc.SampleTime = -1
  offset_llc1_sec_idc.SamplingMode = 'auto'
  offset_llc1_sec_idc.InitialValue = '0'
  offset_llc1_temp_sr = Simulink.Signal
  offset_llc1_temp_sr.DataType = 'uint16'
  offset_llc1_temp_sr.Dimensions = -1
  offset_llc1_temp_sr.DimensionsMode = 'Fixed'
  offset_llc1_temp_sr.Complexity = 'real'
  offset_llc1_temp_sr.SampleTime = -1
  offset_llc1_temp_sr.SamplingMode = 'auto'
  offset_llc1_temp_sr.InitialValue = '1'
  offset_llc2_sec_idc = Simulink.Signal
  offset_llc2_sec_idc.DataType = 'uint16'
  offset_llc2_sec_idc.Dimensions = -1
  offset_llc2_sec_idc.DimensionsMode = 'Fixed'
  offset_llc2_sec_idc.Complexity = 'real'
  offset_llc2_sec_idc.SampleTime = -1
  offset_llc2_sec_idc.SamplingMode = 'auto'
  offset_llc2_sec_idc.InitialValue = '1'
  offset_vbat = Simulink.Signal
  offset_vbat.DataType = 'uint16'
  offset_vbat.Dimensions = -1
  offset_vbat.DimensionsMode = 'Fixed'
  offset_vbat.Complexity = 'real'
  offset_vbat.SampleTime = -1
  offset_vbat.SamplingMode = 'auto'
  offset_vbat.InitialValue = '0'
  offset_vbulk = Simulink.Signal
  offset_vbulk.DataType = 'uint16'
  offset_vbulk.Dimensions = -1
  offset_vbulk.DimensionsMode = 'Fixed'
  offset_vbulk.Complexity = 'real'
  offset_vbulk.SampleTime = -1
  offset_vbulk.SamplingMode = 'auto'
  offset_vbulk.InitialValue = '0'
  offset_vout = Simulink.Signal
  offset_vout.DataType = 'uint16'
  offset_vout.Dimensions = -1
  offset_vout.DimensionsMode = 'Fixed'
  offset_vout.Complexity = 'real'
  offset_vout.SampleTime = -1
  offset_vout.SamplingMode = 'auto'
  offset_vout.InitialValue = '0'
  openloop_en = Simulink.Signal
  openloop_en.DataType = 'boolean'
  openloop_en.Dimensions = -1
  openloop_en.DimensionsMode = 'Fixed'
  openloop_en.Complexity = 'real'
  openloop_en.SampleTime = -1
  openloop_en.SamplingMode = 'auto'
  openloop_en.InitialValue = '0'
  openloop_fault_en = Simulink.Signal
  openloop_fault_en.DataType = 'boolean'
  openloop_fault_en.Dimensions = -1
  openloop_fault_en.DimensionsMode = 'Fixed'
  openloop_fault_en.Complexity = 'real'
  openloop_fault_en.SampleTime = -1
  openloop_fault_en.SamplingMode = 'auto'
  openloop_fault_en.InitialValue = '1'
  ot_fault_120 = Simulink.Signal
  ot_fault_120.DataType = 'boolean'
  ot_fault_120.Dimensions = -1
  ot_fault_120.DimensionsMode = 'Fixed'
  ot_fault_120.Complexity = 'real'
  ot_fault_120.SampleTime = -1
  ot_fault_120.SamplingMode = 'auto'
  ot_fault_120.InitialValue = '0'
  pfc_en = Simulink.Signal
  pfc_en.DataType = 'boolean'
  pfc_en.Dimensions = -1
  pfc_en.DimensionsMode = 'Fixed'
  pfc_en.Complexity = 'real'
  pfc_en.SampleTime = -1
  pfc_en.SamplingMode = 'auto'
  pfc_en.InitialValue = '0'
  pfc_en_120 = Simulink.Signal
  pfc_en_120.DataType = 'boolean'
  pfc_en_120.Dimensions = -1
  pfc_en_120.DimensionsMode = 'Fixed'
  pfc_en_120.Complexity = 'real'
  pfc_en_120.SampleTime = -1
  pfc_en_120.SamplingMode = 'auto'
  pfc_en_120.InitialValue = '0'
  pfc_fw_revision = Simulink.Signal
  pfc_fw_revision.DataType = 'uint16'
  pfc_fw_revision.Dimensions = -1
  pfc_fw_revision.DimensionsMode = 'Fixed'
  pfc_fw_revision.Complexity = 'real'
  pfc_fw_revision.SampleTime = -1
  pfc_fw_revision.SamplingMode = 'auto'
  pfc_fw_revision.InitialValue = '99'
  pfc_fw_revision_bootloader = Simulink.Signal
  pfc_fw_revision_bootloader.DataType = 'uint16'
  pfc_fw_revision_bootloader.Dimensions = -1
  pfc_fw_revision_bootloader.DimensionsMode = 'Fixed'
  pfc_fw_revision_bootloader.Complexity = 'real'
  pfc_fw_revision_bootloader.SampleTime = -1
  pfc_fw_revision_bootloader.SamplingMode = 'auto'
  pfc_fw_revision_bootloader.InitialValue = '99'
  pfc_fw_revision_debug = Simulink.Signal
  pfc_fw_revision_debug.DataType = 'uint16'
  pfc_fw_revision_debug.Dimensions = -1
  pfc_fw_revision_debug.DimensionsMode = 'Fixed'
  pfc_fw_revision_debug.Complexity = 'real'
  pfc_fw_revision_debug.SampleTime = -1
  pfc_fw_revision_debug.SamplingMode = 'auto'
  pfc_fw_revision_debug.InitialValue = '99'
  pfc_ok = Simulink.Signal
  pfc_ok.DataType = 'boolean'
  pfc_ok.Dimensions = -1
  pfc_ok.DimensionsMode = 'Fixed'
  pfc_ok.Complexity = 'real'
  pfc_ok.SampleTime = -1
  pfc_ok.SamplingMode = 'auto'
  pfc_ok.InitialValue = '1'
  pfc_ok_120 = Simulink.Signal
  pfc_ok_120.DataType = 'boolean'
  pfc_ok_120.Dimensions = -1
  pfc_ok_120.DimensionsMode = 'Fixed'
  pfc_ok_120.Complexity = 'real'
  pfc_ok_120.SampleTime = -1
  pfc_ok_120.SamplingMode = 'auto'
  pfc_ok_120.InitialValue = '0'
  pfm_a0 = Simulink.Signal
  pfm_a0.DataType = 'single'
  pfm_a0.Dimensions = -1
  pfm_a0.DimensionsMode = 'Fixed'
  pfm_a0.Complexity = 'real'
  pfm_a0.SampleTime = -1
  pfm_a0.SamplingMode = 'auto'
  pfm_a0.InitialValue = '1'
  pfm_a1 = Simulink.Signal
  pfm_a1.DataType = 'single'
  pfm_a1.Dimensions = -1
  pfm_a1.DimensionsMode = 'Fixed'
  pfm_a1.Complexity = 'real'
  pfm_a1.SampleTime = -1
  pfm_a1.SamplingMode = 'auto'
  pfm_a1.InitialValue = '1'
  pfm_integ_max = Simulink.Signal
  pfm_integ_max.DataType = 'single'
  pfm_integ_max.Dimensions = -1
  pfm_integ_max.DimensionsMode = 'Fixed'
  pfm_integ_max.Complexity = 'real'
  pfm_integ_max.SampleTime = -1
  pfm_integ_max.SamplingMode = 'auto'
  pfm_integ_max.InitialValue = '1'
  pfm_integ_min = Simulink.Signal
  pfm_integ_min.DataType = 'single'
  pfm_integ_min.Dimensions = -1
  pfm_integ_min.DimensionsMode = 'Fixed'
  pfm_integ_min.Complexity = 'real'
  pfm_integ_min.SampleTime = -1
  pfm_integ_min.SamplingMode = 'auto'
  pfm_integ_min.InitialValue = '1'
  pfm_ki = Simulink.Signal
  pfm_ki.DataType = 'single'
  pfm_ki.Dimensions = -1
  pfm_ki.DimensionsMode = 'Fixed'
  pfm_ki.Complexity = 'real'
  pfm_ki.SampleTime = -1
  pfm_ki.SamplingMode = 'auto'
  pfm_ki.InitialValue = '1'
  pfm_kp = Simulink.Signal
  pfm_kp.DataType = 'single'
  pfm_kp.Dimensions = -1
  pfm_kp.DimensionsMode = 'Fixed'
  pfm_kp.Complexity = 'real'
  pfm_kp.SampleTime = -1
  pfm_kp.SamplingMode = 'auto'
  pfm_kp.InitialValue = '1'
  pri_fut_en = Simulink.Signal
  pri_fut_en.DataType = 'uint16'
  pri_fut_en.Dimensions = -1
  pri_fut_en.DimensionsMode = 'Fixed'
  pri_fut_en.Complexity = 'real'
  pri_fut_en.SampleTime = -1
  pri_fut_en.SamplingMode = 'auto'
  pri_fut_en.InitialValue = '99'
  pri_fut_en_buffer = Simulink.Signal
  pri_fut_en_buffer.DataType = 'uint16'
  pri_fut_en_buffer.Dimensions = -1
  pri_fut_en_buffer.DimensionsMode = 'Fixed'
  pri_fut_en_buffer.Complexity = 'real'
  pri_fut_en_buffer.SampleTime = -1
  pri_fut_en_buffer.SamplingMode = 'auto'
  pri_fut_en_buffer.InitialValue = '99'
  pri_halfbridge_en = Simulink.Signal
  pri_halfbridge_en.DataType = 'boolean'
  pri_halfbridge_en.Dimensions = -1
  pri_halfbridge_en.DimensionsMode = 'Fixed'
  pri_halfbridge_en.Complexity = 'real'
  pri_halfbridge_en.SampleTime = -1
  pri_halfbridge_en.SamplingMode = 'auto'
  pri_halfbridge_en.InitialValue = '0'
  pri_halfbridge_en_buffer = Simulink.Signal
  pri_halfbridge_en_buffer.DataType = 'boolean'
  pri_halfbridge_en_buffer.Dimensions = -1
  pri_halfbridge_en_buffer.DimensionsMode = 'Fixed'
  pri_halfbridge_en_buffer.Complexity = 'real'
  pri_halfbridge_en_buffer.SampleTime = -1
  pri_halfbridge_en_buffer.SamplingMode = 'auto'
  pri_halfbridge_en_buffer.InitialValue = '0'
  pspwm_integ_max = Simulink.Signal
  pspwm_integ_max.DataType = 'single'
  pspwm_integ_max.Dimensions = -1
  pspwm_integ_max.DimensionsMode = 'Fixed'
  pspwm_integ_max.Complexity = 'real'
  pspwm_integ_max.SampleTime = -1
  pspwm_integ_max.SamplingMode = 'auto'
  pspwm_integ_max.InitialValue = '1'
  pspwm_integ_min = Simulink.Signal
  pspwm_integ_min.DataType = 'single'
  pspwm_integ_min.Dimensions = -1
  pspwm_integ_min.DimensionsMode = 'Fixed'
  pspwm_integ_min.Complexity = 'real'
  pspwm_integ_min.SampleTime = -1
  pspwm_integ_min.SamplingMode = 'auto'
  pspwm_integ_min.InitialValue = '1'
  pspwm_ki = Simulink.Signal
  pspwm_ki.DataType = 'single'
  pspwm_ki.Dimensions = -1
  pspwm_ki.DimensionsMode = 'Fixed'
  pspwm_ki.Complexity = 'real'
  pspwm_ki.SampleTime = -1
  pspwm_ki.SamplingMode = 'auto'
  pspwm_ki.InitialValue = '-1'
  pspwm_kp = Simulink.Signal
  pspwm_kp.DataType = 'single'
  pspwm_kp.Dimensions = -1
  pspwm_kp.DimensionsMode = 'Fixed'
  pspwm_kp.Complexity = 'real'
  pspwm_kp.SampleTime = -1
  pspwm_kp.SamplingMode = 'auto'
  pspwm_kp.InitialValue = '-1'
  ref_idclink_max = Simulink.Signal
  ref_idclink_max.DataType = 'uint16'
  ref_idclink_max.Dimensions = -1
  ref_idclink_max.DimensionsMode = 'Fixed'
  ref_idclink_max.Complexity = 'real'
  ref_idclink_max.SampleTime = -1
  ref_idclink_max.SamplingMode = 'auto'
  ref_idclink_max.InitialValue = '0'
  ref_iout = Simulink.Signal
  ref_iout.DataType = 'uint16'
  ref_iout.Dimensions = -1
  ref_iout.DimensionsMode = 'Fixed'
  ref_iout.Complexity = 'real'
  ref_iout.SampleTime = -1
  ref_iout.SamplingMode = 'auto'
  ref_iout.InitialValue = '1'
  ref_iout_calib = Simulink.Signal
  ref_iout_calib.DataType = 'uint16'
  ref_iout_calib.Dimensions = -1
  ref_iout_calib.DimensionsMode = 'Fixed'
  ref_iout_calib.Complexity = 'real'
  ref_iout_calib.SampleTime = -1
  ref_iout_calib.SamplingMode = 'auto'
  ref_iout_calib.InitialValue = '99'
  ref_iout_llc1 = Simulink.Signal
  ref_iout_llc1.DataType = 'uint16'
  ref_iout_llc1.Dimensions = -1
  ref_iout_llc1.DimensionsMode = 'Fixed'
  ref_iout_llc1.Complexity = 'real'
  ref_iout_llc1.SampleTime = -1
  ref_iout_llc1.SamplingMode = 'auto'
  ref_iout_llc1.InitialValue = '1'
  ref_iout_llc1_calib = Simulink.Signal
  ref_iout_llc1_calib.DataType = 'uint16'
  ref_iout_llc1_calib.Dimensions = -1
  ref_iout_llc1_calib.DimensionsMode = 'Fixed'
  ref_iout_llc1_calib.Complexity = 'real'
  ref_iout_llc1_calib.SampleTime = -1
  ref_iout_llc1_calib.SamplingMode = 'auto'
  ref_iout_llc1_calib.InitialValue = '334'
  ref_iout_llc2 = Simulink.Signal
  ref_iout_llc2.DataType = 'uint16'
  ref_iout_llc2.Dimensions = -1
  ref_iout_llc2.DimensionsMode = 'Fixed'
  ref_iout_llc2.Complexity = 'real'
  ref_iout_llc2.SampleTime = -1
  ref_iout_llc2.SamplingMode = 'auto'
  ref_iout_llc2.InitialValue = '19'
  ref_iout_llc2_calib = Simulink.Signal
  ref_iout_llc2_calib.DataType = 'uint16'
  ref_iout_llc2_calib.Dimensions = -1
  ref_iout_llc2_calib.DimensionsMode = 'Fixed'
  ref_iout_llc2_calib.Complexity = 'real'
  ref_iout_llc2_calib.SampleTime = -1
  ref_iout_llc2_calib.SamplingMode = 'auto'
  ref_iout_llc2_calib.InitialValue = '300'
  ref_pout = Simulink.Signal
  ref_pout.DataType = 'uint16'
  ref_pout.Dimensions = -1
  ref_pout.DimensionsMode = 'Fixed'
  ref_pout.Complexity = 'real'
  ref_pout.SampleTime = -1
  ref_pout.SamplingMode = 'auto'
  ref_pout.InitialValue = '11000'
  ref_ss_llc1 = Simulink.Signal
  ref_ss_llc1.DataType = 'uint16'
  ref_ss_llc1.Dimensions = -1
  ref_ss_llc1.DimensionsMode = 'Fixed'
  ref_ss_llc1.Complexity = 'real'
  ref_ss_llc1.SampleTime = -1
  ref_ss_llc1.SamplingMode = 'auto'
  ref_ss_llc1.InitialValue = '0'
  ref_ss_llc2 : Simulink.Signal (value not decoded)
  ref_ss_orps : Simulink.Signal (value not decoded)
  ref_vbat : Simulink.Signal (value not decoded)
  ref_vbat_calib : Simulink.Signal (value not decoded)
  ref_vbulk : Simulink.Signal (value not decoded)
  ref_vbulk_calib : Simulink.Signal (value not decoded)
  ref_vbulk_llc1_calib : Simulink.Signal (value not decoded)
  ref_vbulk_llc2_calib : Simulink.Signal (value not decoded)
  ref_vout : Simulink.Signal (value not decoded)
  ref_vout_calib : Simulink.Signal (value not decoded)
  relay_en : Simulink.Signal (value not decoded)
  reset_flag : Simulink.Signal (value not decoded)
  rev_en_120 : Simulink.Signal (value not decoded)
  runtime_control : Simulink.Signal (value not decoded)
  runtime_idle : Simulink.Signal (value not decoded)
  scircv_buffer : Simulink.Signal (value not decoded)
  scircv_buffer_tmp : Simulink.Signal (value not decoded)
  scircv_buffer_tmp_idx0 : Simulink.Signal (value not decoded)
  scircv_chksum : Simulink.Signal (value not decoded)
  scircv_chksum_ok : Simulink.Signal (value not decoded)
  scircv_parse_ok : Simulink.Signal (value not decoded)
  scixmt_buffer : Simulink.Signal (value not decoded)
  scixmt_chksum : Simulink.Signal (value not decoded)
  scixmt_func : Simulink.Signal (value not decoded)
  scixmt_word0_lsb : Simulink.Signal (value not decoded)
  scixmt_word0_msb : Simulink.Signal (value not decoded)
  scixmt_word1_lsb : Simulink.Signal (value not decoded)
  scixmt_word1_msb : Simulink.Signal (value not decoded)
  scixmt_word2_lsb : Simulink.Signal (value not decoded)
  scixmt_word2_msb : Simulink.Signal (value not decoded)
  scixmt_wr : Simulink.Signal (value not decoded)
  ss_step : Simulink.Signal (value not decoded)
  state_calib : Simulink.Signal (value not decoded)
  state_control : Simulink.Signal (value not decoded)
  state_hkeep : Simulink.Signal (value not decoded)
  status_cmpss : Simulink.Signal (value not decoded)
  status_control : Simulink.Signal (value not decoded)
  status_digin : Simulink.Signal (value not decoded)
  status_digout : Simulink.Signal (value not decoded)
  status_fault : Simulink.Signal (value not decoded)
  status_input : Simulink.Signal (value not decoded)
  status_pfc : Simulink.Signal (value not decoded)
  temp_inlet : Simulink.Signal (value not decoded)
  temp_llc1_fet_hs : Simulink.Signal (value not decoded)
  temp_llc2_fet_hs : Simulink.Signal (value not decoded)
  temp_mux : Simulink.Signal (value not decoded)
  temp_mux_s0 : Simulink.Signal (value not decoded)
  temp_mux_s1 : Simulink.Signal (value not decoded)
  temp_mux_s2 : Simulink.Signal (value not decoded)
  temp_outlet : Simulink.Signal (value not decoded)
  temp_pfc_fet_hsa : Simulink.Signal (value not decoded)
  temp_pfc_fet_hsb : Simulink.Signal (value not decoded)
  temp_pfc_fet_hsc : Simulink.Signal (value not decoded)
  temp_pfc_fet_lsa : Simulink.Signal (value not decoded)
  temp_pfc_fet_lsb : Simulink.Signal (value not decoded)
  temp_pfc_fet_lsc : Simulink.Signal (value not decoded)
  test_mode : Simulink.Signal (value not decoded)
  tfcv_cc : Simulink.Signal (value not decoded)
  tfcv_cc_llc2 : Simulink.Signal (value not decoded)
  tfcv_cv : Simulink.Signal (value not decoded)
  tfcv_sr_en : Simulink.Signal (value not decoded)
  tfv_assert_llc1_pri_idc : Simulink.Signal (value not decoded)
  tfv_assert_llc1_sec_idc : Simulink.Signal (value not decoded)
  tfv_assert_llc1_temp_sr : Simulink.Signal (value not decoded)
  tfv_assert_llc2_pri_idc : Simulink.Signal (value not decoded)
  tfv_assert_llc2_sec_idc : Simulink.Signal (value not decoded)
  tfv_assert_llc2_temp_sr : Simulink.Signal (value not decoded)
  tfv_assert_temp_outlet : Simulink.Signal (value not decoded)
  tfv_assert_vaux_uv : Simulink.Signal (value not decoded)
  tfv_assert_vbat : Simulink.Signal (value not decoded)
  tfv_assert_vbulk : Simulink.Signal (value not decoded)
  tfv_assert_vout : Simulink.Signal (value not decoded)
  tfv_cnt_tz : Simulink.Signal (value not decoded)
  tfv_deassert_llc1_pri_idc : Simulink.Signal (value not decoded)
  tfv_deassert_llc1_sec_idc : Simulink.Signal (value not decoded)
  tfv_deassert_llc1_temp_sr : Simulink.Signal (value not decoded)
  tfv_deassert_llc2_pri_idc : Simulink.Signal (value not decoded)
  tfv_deassert_llc2_sec_idc : Simulink.Signal (value not decoded)
  tfv_deassert_llc2_temp_sr : Simulink.Signal (value not decoded)
  tfv_deassert_temp_outlet : Simulink.Signal (value not decoded)
  tfv_deassert_vaux_uv : Simulink.Signal (value not decoded)
  tfv_deassert_vbat : Simulink.Signal (value not decoded)
  tfv_deassert_vbulk : Simulink.Signal (value not decoded)
  tfv_deassert_vout : Simulink.Signal (value not decoded)
  tfv_llc1_pri_idc : Simulink.Signal (value not decoded)
  tfv_llc1_sec_idc : Simulink.Signal (value not decoded)
  tfv_llc1_temp_sr : Simulink.Signal (value not decoded)
  tfv_llc2_pri_idc : Simulink.Signal (value not decoded)
  tfv_llc2_sec_idc : Simulink.Signal (value not decoded)
  tfv_llc2_temp_sr : Simulink.Signal (value not decoded)
  tfv_temp_outlet : Simulink.Signal (value not decoded)
  tfv_vaux_uv : Simulink.Signal (value not decoded)
  tfv_vbat : Simulink.Signal (value not decoded)
  tfv_vbulk : Simulink.Signal (value not decoded)
  tfv_vout : Simulink.Signal (value not decoded)
  timer_1ms : Simulink.Signal (value not decoded)
  tz : Simulink.Signal (value not decoded)
  valve_en : Simulink.Signal (value not decoded)
  vaux : Simulink.Signal (value not decoded)
  vbat : Simulink.Signal (value not decoded)
  vbulk : Simulink.Signal (value not decoded)
  vout : Simulink.Signal (value not decoded)
undefined symbols (not defined in the file or in its folder): CAN_O_INT, CANA_BASE, Down, GPTRIP1SEL, GPTRIP2SEL, TZ1, TZ2, Up
libraries: hdlsllib x159, simulink x94, c2802xlib x32, c2837xDlib x19, c2807xlib x16, c280xlib x13, canmsglib x8, idelinklib_common x2, c2000lib x1, c281xlib x1
(part 1 of 20)
settings Model: DataDictionary=cllc_data_lib.sldd  EnableAccessToBaseWorkspace=off  ExtModeTrigDuration=8  Creator=The MathWorks, Inc.  LastModifiedBy=sgcesuser2
settings SolverCC: AlgebraicLoopSolver=TrustRegion  AutoInsertRateTranBlk=on
settings DataIOCC: LimitDataPoints=on  SaveOutput=off  SaveTime=off  ReturnWorkspaceOutputs=off
settings OptimizationCC: DefaultUnderspecifiedDataType=single  MemcpyThreshold=512  PassReuseOutputArgsAs=Individual arguments  ExpressionDepthLimit=2147483647  LifeSpan=1  MaxStackSize=1024  OptimizeBlockOrder=speed  DifferentSizesBufferReuse=on  DenormalBehavior=FlushToZero  EfficientTunableParamExpr=on
settings DebuggingCC: MergeDetectMultiDrivingBlocksExec=none  SolverPrmCheckMsg=warning  MultiTaskDSMMsg=none  MultiTaskCondExecSysMsg=none  FcnCallInpInsideContextMsg=warning  UnconnectedInputMsg=warning  UnconnectedOutputMsg=warning  UnconnectedLineMsg=warning  AllowSymbolicDim=off  StateNameClashWarn=warning  SFUnexpectedBacktrackingDiag=warning  SFNoUnconditionalDefaultTransitionDiag=warning  SFExecutionAtInitializationDiag=none  SFMachineParentedDataDiag=warning  ArithmeticOperatorsInVariantConditions=warning
settings HardwareCC: ProdBitPerChar=16  ProdBitPerInt=16  ProdBitPerPointer=32  ProdBitPerSizeT=32  ProdBitPerPtrDiffT=32  ProdLargestAtomicInteger=Integer  ProdLargestAtomicFloat=None  ProdWordSize=16  ProdLongLongMode=on  ProdHWDeviceType=Texas Instruments->C2000
settings ModelReferenceCC: PropagateSignalLabelsOutOfModel=off
settings SFSimCC: SimUseLocalCustomCode=off  SimParseCustomCode=off  MATLABDynamicMemAlloc=off  CustomCodeUndefinedFunction=UseInterfaceOnly
settings RTWCC: SystemTargetFile=ert.tlc  HardwareBoard=TI Delfino F2837xS  TemplateMakefile=ert_default_tmf  GenerateReport=on  RTWUseLocalCustomCode=off  Toolchain=Texas Instruments Code Composer Studio (C2000)  IncludeHyperlinkInReport=on  LaunchReport=on  GenerateTraceInfo=on  GenerateTraceReport=on  GenerateTraceReportSl=on  GenerateTraceReportSf=on  GenerateTraceReportEml=on  GenerateCodeMetricsReport=on  DLArmComputeVersion=19.05
settings RTWCC: CustomHeaderCode=|
  | //#include "adc.h"
  | #include "asysctl.h"
  | //#include "can.h"
  | #include "cla.h"
  | #include "cmpss.h"
  | #include "cpu.h"
  | #include "cputimer.h"
  | #include "dac.h"
  | #include "dcsm.h"
  | #include "debug.h"
  | #include "dma.h"
  | #include "ecap.h"
  | #include "emif.h"
  | #include "epwm.h"
  | #include "eqep.h"
  | #include "flash.h"
  | #include "gpio.h"
  | #include "hrpwm.h"
  | #include "i2c.h"
  | #include "interrupt.h"
  | #include "mcbsp.h"
  | #include "memcfg.h"
  | #include "pin_map.h"
  | #include "sci.h"
  | #include "sdfm.h"
  | #include "spi.h"
  | #include "sysctl.h"
  | //#include "upp.h"
  | #include "version.h"
  | #include "xbar.h"
  | #include "clb.h"
  | #include "clb_config.h"
settings RTWCC: CustomInclude=|
  | C:\ti\C2000\C2000Ware_4_00_00_00\driverlib\f2837xs\driverlib
  | C:\ti\C2000\C2000Ware_4_00_00_00\device_support\f2837xs\common\include
settings RTWCC: CustomSource=|
  | C:\ti\C2000\C2000Ware_4_00_00_00\driverlib\f2837xs\driverlib\cmpss.c
  | C:\ti\C2000\C2000Ware_4_00_00_00\driverlib\f2837xs\driverlib\xbar.c
  | C:\ti\C2000\C2000Ware_4_00_00_00\driverlib\f2837xs\driverlib\gpio.c
  | C:\ti\C2000\C2000Ware_4_00_00_00\driverlib\f2837xs\driverlib\clb.c
  | clb_config.c
settings CodeAppCC: IgnoreCustomStorageClasses=off  CustomSymbolStrType=$N$R$M  CustomSymbolStrFcn=$N$M$F  CustomSymbolStrModelFcn=$N  StateflowObjectComments=on  InternalIdentifier=Classic
settings ERTTargetCC: CodeReplacementLibrary=TI C28x  MultiwordLength=2048  SupportNonInlinedSFcns=on  ExtModeTransport=4  ExtModeStaticAlloc=on  ExtModeStaticAllocSize=2000  ExtModeMexFile=ext_xcp  ExtModeIntrfLevel=Level2 - Open  ConvertIfToSwitch=off  SuppressUnreachableDefaultCases=off
settings ConfigComp: CovMetricSettings=dw  CovSaveCumulativeToWorkspaceVar=on  CovSaveSingleToWorkspaceVar=on  CovExternalEMLEnable=off  CovSFcnEnable=off

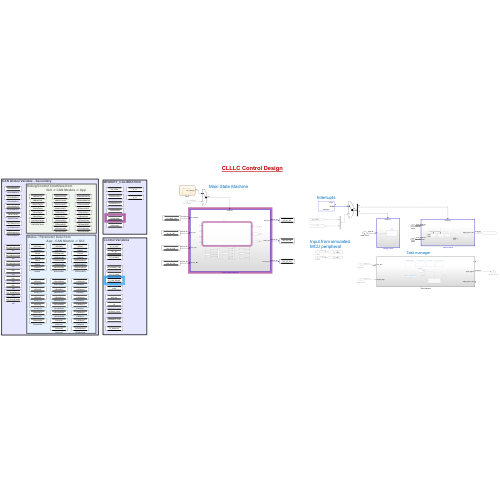
[thumbnail: Simulink's stored preview of the top-level diagram]
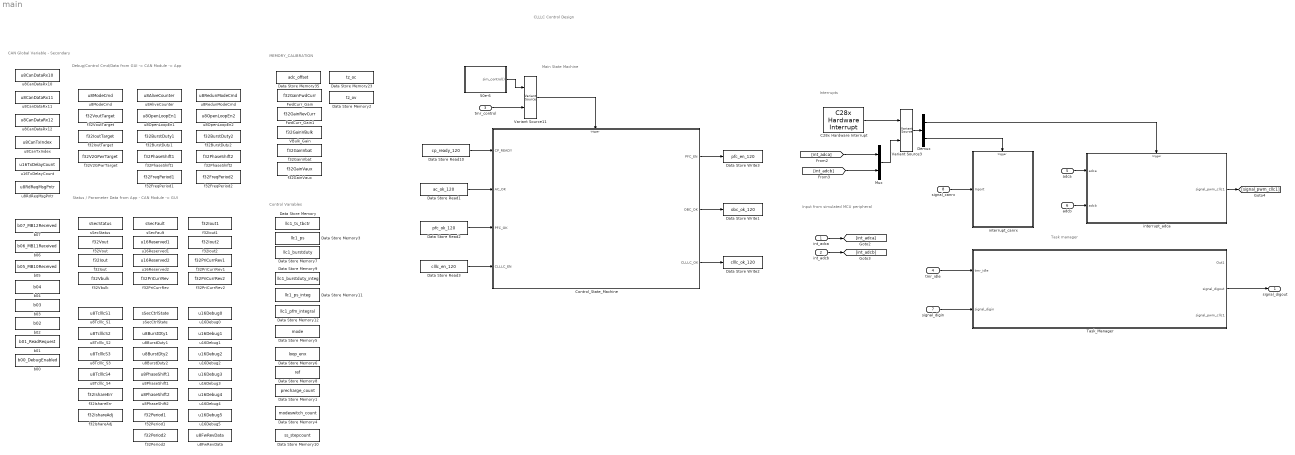
== system main ==
  note: Task manager
  note: CLLLC Control Design
  note: Interrupts
  note: Main State Machine
  note: Input from simulated
      | MCU peripheral
  note: CAN Global Variable - Secondary
  note: Debug/Control Cmd/Data from
      |                       GUI -> CAN Module -> App
  note: Status / Parameter Data from
      |                       App - CAN Module -> GUI
  note: MEMORY_CALIBRATION
  note: Control Variables
  int_adca : Inport  OutputFunctionCall=on
  int_adcb : Inport  Port=2  OutputFunctionCall=on
  tmr_control : Inport  Port=3  OutputFunctionCall=on
  tmr_idle : Inport  Port=4  OutDataTypeStr=single  OutputFunctionCall=on
  adca : Inport  Port=5  OutDataTypeStr=Bus: adca_digital  BusOutputAsStruct=on
  adcb : Inport  Port=6  OutDataTypeStr=Bus: adcb_digital  BusOutputAsStruct=on
  signal_digin : Inport  Port=7
  signal_canrx : Inport  Port=8
  50e-6 : Stateflow chart  TreatAsAtomicUnit=on  SystemSampleTime=50e-6
  C28x Hardware Interrupt : c2000lib/Scheduling/C28x Hardware Interrupt  irqnumbers=[1 9]  pienumbers=[1 5]  irqpriorities=[30 31]  irqpreempts=[0 1]  showinput=off  dspchiptype=C280X
      settings: SourceProductBaseCode=TIC2000
  Control_State_Machine : Subsystem
  Data Store Memory : DataStoreMemory  DataStoreName=llc1_ts_tbctr  ReadBeforeWriteMsg=warning  WriteAfterWriteMsg=warning  WriteAfterReadMsg=warning  InitialValue=1000  EmbeddedSignalClassName=tic2000demospkg.Signal  ShowAdditionalParam=off  OutDataTypeStr=single
  Data Store Memory1 : DataStoreMemory  DataStoreName=precharge_count  ReadBeforeWriteMsg=warning  WriteAfterWriteMsg=warning  WriteAfterReadMsg=warning  ShowAdditionalParam=off  OutDataTypeStr=uint16
  Data Store Memory10 : DataStoreMemory  DataStoreName=ss_stepcount  WriteAfterWriteMsg=warning  ShowAdditionalParam=off  OutDataTypeStr=uint16
  Data Store Memory11 : DataStoreMemory  DataStoreName=llc1_ps_integ  ReadBeforeWriteMsg=warning  WriteAfterWriteMsg=warning  WriteAfterReadMsg=warning  ShowAdditionalParam=off  OutDataTypeStr=single
  Data Store Memory12 : DataStoreMemory  DataStoreName=llc1_pfm_integral  ReadBeforeWriteMsg=warning  WriteAfterWriteMsg=warning  WriteAfterReadMsg=warning  ShowAdditionalParam=off  OutDataTypeStr=single
  Data Store Memory2 : DataStoreMemory  DataStoreName=tz_ov  ReadBeforeWriteMsg=warning  WriteAfterWriteMsg=warning  WriteAfterReadMsg=warning  ShowAdditionalParam=off  OutDataTypeStr=uint16
  Data Store Memory23 : DataStoreMemory  DataStoreName=tz_oc  ReadBeforeWriteMsg=warning  WriteAfterWriteMsg=warning  WriteAfterReadMsg=warning  ShowAdditionalParam=off  OutDataTypeStr=uint16
  Data Store Memory3 : DataStoreMemory  DataStoreName=llc1_ps  ReadBeforeWriteMsg=warning  WriteAfterWriteMsg=warning  WriteAfterReadMsg=warning  InitialValue=36  EmbeddedSignalClassName=tic2000demospkg.Signal  ShowAdditionalParam=off  OutDataTypeStr=single
  Data Store Memory35 : DataStoreMemory  DataStoreName=adc_offset  ReadBeforeWriteMsg=warning  WriteAfterWriteMsg=warning  WriteAfterReadMsg=warning  ShowAdditionalParam=off  OutDataTypeStr=single
  Data Store Memory4 : DataStoreMemory  DataStoreName=modeswitch_count  ReadBeforeWriteMsg=warning  WriteAfterWriteMsg=warning  WriteAfterReadMsg=warning  ShowAdditionalParam=off  OutDataTypeStr=uint16
  Data Store Memory5 : DataStoreMemory  DataStoreName=mode  ReadBeforeWriteMsg=warning  WriteAfterWriteMsg=warning  WriteAfterReadMsg=warning  ShowAdditionalParam=off  OutDataTypeStr=uint16
  Data Store Memory6 : DataStoreMemory  DataStoreName=loop_enx  ReadBeforeWriteMsg=warning  WriteAfterWriteMsg=warning  WriteAfterReadMsg=warning  ShowAdditionalParam=off  OutDataTypeStr=uint16
  Data Store Memory7 : DataStoreMemory  DataStoreName=llc1_burstduty  ReadBeforeWriteMsg=warning  WriteAfterWriteMsg=warning  WriteAfterReadMsg=warning  EmbeddedSignalClassName=tic2000demospkg.Signal  ShowAdditionalParam=off  OutDataTypeStr=single
  Data Store Memory8 : DataStoreMemory  DataStoreName=ref  ReadBeforeWriteMsg=warning  WriteAfterWriteMsg=warning  WriteAfterReadMsg=warning  ShowAdditionalParam=off  OutDataTypeStr=uint16
  Data Store Memory9 : DataStoreMemory  DataStoreName=llc1_burstduty_integ  ReadBeforeWriteMsg=warning  WriteAfterWriteMsg=warning  WriteAfterReadMsg=warning  ShowAdditionalParam=off  OutDataTypeStr=single
  Data Store Read1 : DataStoreRead  DataStoreName=ac_ok_120  IndexOptions=Index vector (dialog)  Indices=1  OutputSizes=1
  Data Store Read10 : DataStoreRead  DataStoreName=cp_ready_120  IndexOptions=Index vector (dialog)  Indices=1  OutputSizes=1
  Data Store Read2 : DataStoreRead  DataStoreName=pfc_ok_120  IndexOptions=Index vector (dialog)  Indices=1  OutputSizes=1
  Data Store Read3 : DataStoreRead  DataStoreName=clllc_en_120  IndexOptions=Index vector (dialog)  Indices=1  OutputSizes=1
  Data Store Write1 : DataStoreWrite  DataStoreName=obc_ok_120  IndexOptions=Index vector (dialog)  Indices=1  OutputSizes=1
  Data Store Write2 : DataStoreWrite  DataStoreName=clllc_ok_120  IndexOptions=Index vector (dialog)  Indices=1  OutputSizes=1
  Data Store Write3 : DataStoreWrite  DataStoreName=pfc_en_120  IndexOptions=Index vector (dialog)  Indices=1  OutputSizes=1
  Demux : Demux  Outputs=2
  FwdCurr_Gain : DataStoreMemory  DataStoreName=f32GainFwdCurr  ReadBeforeWriteMsg=warning  WriteAfterWriteMsg=warning  WriteAfterReadMsg=warning  InitialValue=(3.3/4095)*(1/0.02)  ShowAdditionalParam=off  OutDataTypeStr=single
  FwdCurr_Gain1 : DataStoreMemory  DataStoreName=f32GainRevCurr  ReadBeforeWriteMsg=warning  WriteAfterWriteMsg=warning  WriteAfterReadMsg=warning  InitialValue=(3.3/4095)*(1/0.02)  ShowAdditionalParam=off  OutDataTypeStr=single
  Mux : Mux  Inputs=2
  Task_Manager : Subsystem
  VBulk_Gain : DataStoreMemory  DataStoreName=f32GainVBulk  ReadBeforeWriteMsg=warning  WriteAfterWriteMsg=warning  WriteAfterReadMsg=warning  InitialValue=(3.3/4095)*(1/0.00272)  ShowAdditionalParam=off  OutDataTypeStr=single
  Variant Source11 : VariantSource
      settings: AllowZeroVariantControls=on
  Variant Source3 : VariantSource
      settings: AllowZeroVariantControls=on
  b00 : DataStoreMemory  DataStoreName=b00_DebugEnabled  ReadBeforeWriteMsg=warning  WriteAfterWriteMsg=warning  WriteAfterReadMsg=warning  ShowAdditionalParam=off  OutDataTypeStr=boolean
  b01 : DataStoreMemory  DataStoreName=b01_ReadRequest  ReadBeforeWriteMsg=warning  WriteAfterWriteMsg=warning  WriteAfterReadMsg=warning  ShowAdditionalParam=off  OutDataTypeStr=boolean
  b02 : DataStoreMemory  DataStoreName=b02  ReadBeforeWriteMsg=warning  WriteAfterWriteMsg=warning  WriteAfterReadMsg=warning  ShowAdditionalParam=off  OutDataTypeStr=boolean
  b03 : DataStoreMemory  DataStoreName=b03  ReadBeforeWriteMsg=warning  WriteAfterWriteMsg=warning  WriteAfterReadMsg=warning  ShowAdditionalParam=off  OutDataTypeStr=boolean
  b04 : DataStoreMemory  DataStoreName=b04  ReadBeforeWriteMsg=warning  WriteAfterWriteMsg=warning  WriteAfterReadMsg=warning  ShowAdditionalParam=off  OutDataTypeStr=boolean
  b05 : DataStoreMemory  DataStoreName=b05_MB10Received  ReadBeforeWriteMsg=warning  WriteAfterWriteMsg=warning  WriteAfterReadMsg=warning  ShowAdditionalParam=off  OutDataTypeStr=boolean
  b06 : DataStoreMemory  DataStoreName=b06_MB11Received  ReadBeforeWriteMsg=warning  WriteAfterWriteMsg=warning  WriteAfterReadMsg=warning  ShowAdditionalParam=off  OutDataTypeStr=boolean
  b07 : DataStoreMemory  DataStoreName=b07_MB12Received  ReadBeforeWriteMsg=warning  WriteAfterWriteMsg=warning  WriteAfterReadMsg=warning  ShowAdditionalParam=off  OutDataTypeStr=boolean
  f32BurstDuty1 : DataStoreMemory  DataStoreName=f32BurstDuty1  ReadBeforeWriteMsg=warning  WriteAfterWriteMsg=warning  WriteAfterReadMsg=warning  InitialValue=100  ShowAdditionalParam=off  OutDataTypeStr=single
  f32BurstDuty2 : DataStoreMemory  DataStoreName=f32BurstDuty2  ReadBeforeWriteMsg=warning  WriteAfterWriteMsg=warning  WriteAfterReadMsg=warning  InitialValue=100  ShowAdditionalParam=off  OutDataTypeStr=single
  f32FreqPeriod1 : DataStoreMemory  DataStoreName=f32FreqPeriod1  ReadBeforeWriteMsg=warning  WriteAfterWriteMsg=warning  WriteAfterReadMsg=warning  InitialValue=1000  ShowAdditionalParam=off  OutDataTypeStr=single
  f32FreqPeriod2 : DataStoreMemory  DataStoreName=f32FreqPeriod2  ReadBeforeWriteMsg=warning  WriteAfterWriteMsg=warning  WriteAfterReadMsg=warning  InitialValue=300  ShowAdditionalParam=off  OutDataTypeStr=single
  f32GainVaux : DataStoreMemory  DataStoreName=f32GainVaux  ReadBeforeWriteMsg=warning  WriteAfterWriteMsg=warning  WriteAfterReadMsg=warning  InitialValue=(3.3/4095)*(1/0.20325)  ShowAdditionalParam=off  OutDataTypeStr=single
  f32GainVbat : DataStoreMemory  DataStoreName=f32GainVbat  ReadBeforeWriteMsg=warning  WriteAfterWriteMsg=warning  WriteAfterReadMsg=warning  InitialValue=(3.3/4095)*(1/0.00569)  ShowAdditionalParam=off  OutDataTypeStr=single
  f32Iout : DataStoreMemory  DataStoreName=f32Iout  ReadBeforeWriteMsg=warning  WriteAfterWriteMsg=warning  WriteAfterReadMsg=warning  ShowAdditionalParam=off  OutDataTypeStr=single
  f32Iout1 : DataStoreMemory  DataStoreName=f32Iout1  ReadBeforeWriteMsg=warning  WriteAfterWriteMsg=warning  WriteAfterReadMsg=warning  ShowAdditionalParam=off  OutDataTypeStr=single
  f32Iout2 : DataStoreMemory  DataStoreName=f32Iout2  ReadBeforeWriteMsg=warning  WriteAfterWriteMsg=warning  WriteAfterReadMsg=warning  ShowAdditionalParam=off  OutDataTypeStr=single
  f32IoutTarget : DataStoreMemory  DataStoreName=f32IoutTarget  ReadBeforeWriteMsg=warning  WriteAfterWriteMsg=warning  WriteAfterReadMsg=warning  InitialValue=1  ShowAdditionalParam=off  OutDataTypeStr=single
  f32IshareAdj : DataStoreMemory  DataStoreName=f32IshareAdj  ReadBeforeWriteMsg=warning  WriteAfterWriteMsg=warning  WriteAfterReadMsg=warning  ShowAdditionalParam=off  OutDataTypeStr=single
  f32IshareErr : DataStoreMemory  DataStoreName=f32IshareErr  ReadBeforeWriteMsg=warning  WriteAfterWriteMsg=warning  WriteAfterReadMsg=warning  ShowAdditionalParam=off  OutDataTypeStr=single
  f32Period1 : DataStoreMemory  DataStoreName=f32Period1  ReadBeforeWriteMsg=warning  WriteAfterWriteMsg=warning  WriteAfterReadMsg=warning  ShowAdditionalParam=off  OutDataTypeStr=single
  f32Period2 : DataStoreMemory  DataStoreName=f32Period2  ReadBeforeWriteMsg=warning  WriteAfterWriteMsg=warning  WriteAfterReadMsg=warning  ShowAdditionalParam=off  OutDataTypeStr=single
  f32PhaseShift1 : DataStoreMemory  DataStoreName=f32PhaseShift1  ReadBeforeWriteMsg=warning  WriteAfterWriteMsg=warning  WriteAfterReadMsg=warning  ShowAdditionalParam=off  OutDataTypeStr=single
  f32PhaseShift2 : DataStoreMemory  DataStoreName=f32PhaseShift2  ReadBeforeWriteMsg=warning  WriteAfterWriteMsg=warning  WriteAfterReadMsg=warning  InitialValue=100  ShowAdditionalParam=off  OutDataTypeStr=single
  f32PriCurrRev : DataStoreMemory  DataStoreName=f32PriCurrRev  ReadBeforeWriteMsg=warning  WriteAfterWriteMsg=warning  WriteAfterReadMsg=warning  ShowAdditionalParam=off  OutDataTypeStr=single
  f32PriCurrRev1 : DataStoreMemory  DataStoreName=f32PriCurrRev1  ReadBeforeWriteMsg=warning  WriteAfterWriteMsg=warning  WriteAfterReadMsg=warning  ShowAdditionalParam=off  OutDataTypeStr=single
  f32PriCurrRev2 : DataStoreMemory  DataStoreName=f32PriCurrRev2  ReadBeforeWriteMsg=warning  WriteAfterWriteMsg=warning  WriteAfterReadMsg=warning  ShowAdditionalParam=off  OutDataTypeStr=single
  f32V2GPwrTarget : DataStoreMemory  DataStoreName=f32V2GPwrTarget  ReadBeforeWriteMsg=warning  WriteAfterWriteMsg=warning  WriteAfterReadMsg=warning  InitialValue=0.0  ShowAdditionalParam=off  OutDataTypeStr=single
  f32Vbulk : DataStoreMemory  DataStoreName=f32Vbulk  ReadBeforeWriteMsg=warning  WriteAfterWriteMsg=warning  WriteAfterReadMsg=warning  ShowAdditionalParam=off  OutDataTypeStr=single
  f32Vout : DataStoreMemory  DataStoreName=f32Vout  ReadBeforeWriteMsg=warning  WriteAfterWriteMsg=warning  WriteAfterReadMsg=warning  ShowAdditionalParam=off  OutDataTypeStr=single
  f32VoutTarget : DataStoreMemory  DataStoreName=f32VoutTarget  ReadBeforeWriteMsg=warning  WriteAfterWriteMsg=warning  WriteAfterReadMsg=warning  InitialValue=250  ShowAdditionalParam=off  OutDataTypeStr=single
  interrupt_adca : Subsystem  TreatAsAtomicUnit=on
      settings: RTWFcnNameOpts=Use subsystem name  RTWFileNameOpts=Use subsystem name
  interrupt_canrx : Subsystem  TreatAsAtomicUnit=on
      settings: RTWFcnNameOpts=Use subsystem name  RTWFileNameOpts=Use subsystem name
  sSecCtrlState : DataStoreMemory  DataStoreName=sSecCtrlState  ReadBeforeWriteMsg=warning  WriteAfterWriteMsg=warning  WriteAfterReadMsg=warning  ShowAdditionalParam=off  OutDataTypeStr=uint8
  sSecFault : DataStoreMemory  DataStoreName=sSecFault  ReadBeforeWriteMsg=warning  WriteAfterWriteMsg=warning  WriteAfterReadMsg=warning  ShowAdditionalParam=off  OutDataTypeStr=uint16
  sSecStatus : DataStoreMemory  DataStoreName=sSecStatus  ReadBeforeWriteMsg=warning  WriteAfterWriteMsg=warning  WriteAfterReadMsg=warning  ShowAdditionalParam=off  OutDataTypeStr=uint16
  u16Debug0 : DataStoreMemory  DataStoreName=u16Debug0  ReadBeforeWriteMsg=warning  WriteAfterWriteMsg=warning  WriteAfterReadMsg=warning  ShowAdditionalParam=off  OutDataTypeStr=uint16
  u16Debug1 : DataStoreMemory  DataStoreName=u16Debug1  ReadBeforeWriteMsg=warning  WriteAfterWriteMsg=warning  WriteAfterReadMsg=warning  ShowAdditionalParam=off  OutDataTypeStr=uint16
  u16Debug2 : DataStoreMemory  DataStoreName=u16Debug2  ReadBeforeWriteMsg=warning  WriteAfterWriteMsg=warning  WriteAfterReadMsg=warning  ShowAdditionalParam=off  OutDataTypeStr=uint16
  u16Debug3 : DataStoreMemory  DataStoreName=u16Debug3  ReadBeforeWriteMsg=warning  WriteAfterWriteMsg=warning  WriteAfterReadMsg=warning  ShowAdditionalParam=off  OutDataTypeStr=uint16
  u16Debug4 : DataStoreMemory  DataStoreName=u16Debug4  ReadBeforeWriteMsg=warning  WriteAfterWriteMsg=warning  WriteAfterReadMsg=warning  ShowAdditionalParam=off  OutDataTypeStr=uint16
  u16Debug5 : DataStoreMemory  DataStoreName=u16Debug5  ReadBeforeWriteMsg=warning  WriteAfterWriteMsg=warning  WriteAfterReadMsg=warning  ShowAdditionalParam=off  OutDataTypeStr=uint16
  u16Reserved1 : DataStoreMemory  DataStoreName=u16Reserved1  ReadBeforeWriteMsg=warning  WriteAfterWriteMsg=warning  WriteAfterReadMsg=warning  ShowAdditionalParam=off  OutDataTypeStr=uint16
  u16Reserved2 : DataStoreMemory  DataStoreName=u16Reserved2  ReadBeforeWriteMsg=warning  WriteAfterWriteMsg=warning  WriteAfterReadMsg=warning  ShowAdditionalParam=off  OutDataTypeStr=uint16
  u16TxDelayCount : DataStoreMemory  DataStoreName=u16TxDelayCount  ReadBeforeWriteMsg=warning  WriteAfterWriteMsg=warning  WriteAfterReadMsg=warning  ShowAdditionalParam=off  OutDataTypeStr=uint16
  u8AliveCounter : DataStoreMemory  DataStoreName=u8AliveCounter  ReadBeforeWriteMsg=warning  WriteAfterWriteMsg=warning  WriteAfterReadMsg=warning  ShowAdditionalParam=off  OutDataTypeStr=uint8
  u8BurstDuty1 : DataStoreMemory  DataStoreName=u8BurstDty1  ReadBeforeWriteMsg=warning  WriteAfterWriteMsg=warning  WriteAfterReadMsg=warning  ShowAdditionalParam=off  OutDataTypeStr=uint8
  u8BurstDuty2 : DataStoreMemory  DataStoreName=u8BurstDty2  ReadBeforeWriteMsg=warning  WriteAfterWriteMsg=warning  WriteAfterReadMsg=warning  ShowAdditionalParam=off  OutDataTypeStr=uint8
  u8CanDataRx10 : DataStoreMemory  DataStoreName=u8CanDataRx10  ReadBeforeWriteMsg=warning  WriteAfterWriteMsg=warning  WriteAfterReadMsg=warning  InitialValue=[0 0 0 0 0 0 0 0]  ShowAdditionalParam=off  OutDataTypeStr=uint8  Dimensions=[8 1]
  u8CanDataRx11 : DataStoreMemory  DataStoreName=u8CanDataRx11  ReadBeforeWriteMsg=warning  WriteAfterWriteMsg=warning  WriteAfterReadMsg=warning  InitialValue=[0 0 0 0 0 0 0 0]  ShowAdditionalParam=off  OutDataTypeStr=uint8  Dimensions=[8 1]
  u8CanDataRx12 : DataStoreMemory  DataStoreName=u8CanDataRx12  ReadBeforeWriteMsg=warning  WriteAfterWriteMsg=warning  WriteAfterReadMsg=warning  InitialValue=[0 0 0 0 0 0 0 0]  ShowAdditionalParam=off  OutDataTypeStr=uint8  Dimensions=[8 1]
  u8CanTxIndex : DataStoreMemory  DataStoreName=u8CanTxIndex  ReadBeforeWriteMsg=warning  WriteAfterWriteMsg=warning  WriteAfterReadMsg=warning  ShowAdditionalParam=off  OutDataTypeStr=uint8
  u8FwRevData : DataStoreMemory  DataStoreName=u8FwRevData  ReadBeforeWriteMsg=warning  WriteAfterWriteMsg=warning  WriteAfterReadMsg=warning  InitialValue=[0 0 0 0 0 0 0 0]  ShowAdditionalParam=off  OutDataTypeStr=uint8  Dimensions=[8 1]
  u8ModeCmd : DataStoreMemory  DataStoreName=u8ModeCmd  ReadBeforeWriteMsg=warning  WriteAfterWriteMsg=warning  WriteAfterReadMsg=warning  InitialValue=160  ShowAdditionalParam=off  OutDataTypeStr=uint8
  u8OpenLoopEn1 : DataStoreMemory  DataStoreName=u8OpenLoopEn1  ReadBeforeWriteMsg=warning  WriteAfterWriteMsg=warning  WriteAfterReadMsg=warning  ShowAdditionalParam=off  OutDataTypeStr=uint8
  u8OpenLoopEn2 : DataStoreMemory  DataStoreName=u8OpenLoopEn2  ReadBeforeWriteMsg=warning  WriteAfterWriteMsg=warning  WriteAfterReadMsg=warning  ShowAdditionalParam=off  OutDataTypeStr=uint8
  u8PhaseShift1 : DataStoreMemory  DataStoreName=u8PhaseShift1  ReadBeforeWriteMsg=warning  WriteAfterWriteMsg=warning  WriteAfterReadMsg=warning  ShowAdditionalParam=off  OutDataTypeStr=uint8
  u8PhaseShift2 : DataStoreMemory  DataStoreName=u8PhaseShift2  ReadBeforeWriteMsg=warning  WriteAfterWriteMsg=warning  WriteAfterReadMsg=warning  ShowAdditionalParam=off  OutDataTypeStr=uint8
  u8RdReqMsgPntr : DataStoreMemory  DataStoreName=u8RdReqMsgPntr  ReadBeforeWriteMsg=warning  WriteAfterWriteMsg=warning  WriteAfterReadMsg=warning  ShowAdditionalParam=off  OutDataTypeStr=uint8
  u8RedunModeCmd : DataStoreMemory  DataStoreName=u8RedunModeCmd  ReadBeforeWriteMsg=warning  WriteAfterWriteMsg=warning  WriteAfterReadMsg=warning  ShowAdditionalParam=off  OutDataTypeStr=uint8
  u8Tclllc_S1 : DataStoreMemory  DataStoreName=u8TclllcS1  ReadBeforeWriteMsg=warning  WriteAfterWriteMsg=warning  WriteAfterReadMsg=warning  ShowAdditionalParam=off  OutDataTypeStr=uint8
  u8Tclllc_S2 : DataStoreMemory  DataStoreName=u8TclllcS2  ReadBeforeWriteMsg=warning  WriteAfterWriteMsg=warning  WriteAfterReadMsg=warning  ShowAdditionalParam=off  OutDataTypeStr=uint8
  u8Tclllc_S3 : DataStoreMemory  DataStoreName=u8TclllcS3  ReadBeforeWriteMsg=warning  WriteAfterWriteMsg=warning  WriteAfterReadMsg=warning  ShowAdditionalParam=off  OutDataTypeStr=uint8
  u8Tclllc_S4 : DataStoreMemory  DataStoreName=u8TclllcS4  ReadBeforeWriteMsg=warning  WriteAfterWriteMsg=warning  WriteAfterReadMsg=warning  ShowAdditionalParam=off  OutDataTypeStr=uint8
  signal_digout : Outport
  wires:
  C28x Hardware Interrupt/1 -> Variant Source3/1
  adca/1 -> interrupt_adca/1(adca)
  Variant Source3/1 -> Demux/1
  adcb/1 -> interrupt_adca/2(adcb)
  Variant Source11/1 -> Control_State_Machine/Trigger
  50e-6/1(sim_control()) -> Variant Source11/1
  Mux/1 -> Variant Source3/2
  int_adca/1 -> [int_adca]
  int_adcb/1 -> [int_adcb]
  [int_adca] -> Mux/1
  [int_adcb] -> Mux/2
  tmr_control/1 -> Variant Source11/2
  Demux/1 -> interrupt_adca/Trigger
  Demux/2 -> interrupt_canrx/Trigger
  signal_digin/1 -> Task_Manager/2(signal_digin)
  Task_Manager/2(signal_digout) -> signal_digout/1
  interrupt_adca/1(signal_pwm_cllc1) -> [signal_pwm_cllc1]
  signal_canrx/1 -> interrupt_canrx/1(Inport)
  tmr_idle/1 -> Task_Manager/1(tmr_idle)
  Data Store Read3/1 -> Control_State_Machine/4(CLLLC_EN)
  Data Store Read10/1 -> Control_State_Machine/1(CP_READY)
  Data Store Read1/1 -> Control_State_Machine/2(AC_OK)
  Data Store Read2/1 -> Control_State_Machine/3(PFC_OK)
  Control_State_Machine/1(PFC_EN) -> Data Store Write3/1
  Control_State_Machine/2(OBC_OK) -> Data Store Write1/1
  Control_State_Machine/3(CLLLC_OK) -> Data Store Write2/1

== system main/Control_State_Machine ==
  CP_READY : Inport
  AC_OK : Inport  Port=2
  PFC_OK : Inport  Port=3
  CLLLC_EN : Inport  Port=4
  function : TriggerPort  TriggerType=function-call  VariantControl=Variant
  Control diagnostics : Scope  NumInputPorts=4
  Data Store Read : DataStoreRead  DataStoreName=llc1_ts_tbctr  IndexOptions=Index vector (dialog)  Indices=1  OutputSizes=1
  Data Store Read1 : DataStoreRead  DataStoreName=llc1_ps  IndexOptions=Index vector (dialog)  Indices=1  OutputSizes=1
  Data Store Read12 : DataStoreRead  DataStoreName=ref_vout_calib  IndexOptions=Index vector (dialog)  Indices=1  OutputSizes=1
  Data Store Read13 : DataStoreRead  DataStoreName=vout  IndexOptions=Index vector (dialog)  Indices=1  OutputSizes=1
  Data Store Read14 : DataStoreRead  DataStoreName=mode  IndexOptions=Index vector (dialog)  Indices=1  OutputSizes=1
  Data Store Read2 : DataStoreRead  DataStoreName=llc1_burstduty  IndexOptions=Index vector (dialog)  Indices=1  OutputSizes=1
  Data Store Read3 : DataStoreRead  DataStoreName=mode  IndexOptions=Index vector (dialog)  Indices=1  OutputSizes=1
  Data Store Read4 : DataStoreRead  DataStoreName=ref_iout_llc1_calib  IndexOptions=Index vector (dialog)  Indices=1  OutputSizes=1
  Data Store Read5 : DataStoreRead  DataStoreName=llc1_sec_idc  IndexOptions=Index vector (dialog)  Indices=1  OutputSizes=1
  Data Store Read6 : DataStoreRead  DataStoreName=ref_vbulk_calib  IndexOptions=Index vector (dialog)  Indices=1  OutputSizes=1
  Data Store Read7 : DataStoreRead  DataStoreName=vbulk  IndexOptions=Index vector (dialog)  Indices=1  OutputSizes=1
  Data Store Read8 : DataStoreRead  DataStoreName=mode  IndexOptions=Index vector (dialog)  Indices=1  OutputSizes=1
  Data Type Conversion : DataTypeConversion  OutDataTypeStr=boolean  SaturateOnIntegerOverflow=off  RndMeth=Floor
  Data Type Conversion1 : DataTypeConversion  OutDataTypeStr=boolean  SaturateOnIntegerOverflow=off  RndMeth=Floor
  Data Type Conversion2 : DataTypeConversion  OutDataTypeStr=boolean  SaturateOnIntegerOverflow=off  RndMeth=Floor
  Multiply : Gain  Gain=200
  Ref_fbk_fwd : Scope  NumInputPorts=5
  Ref_fbk_rev : Scope  NumInputPorts=3
  control : Stateflow chart  TreatAsAtomicUnit=on
  PFC_EN : Outport
  OBC_OK : Outport  Port=2
  CLLLC_OK : Outport  Port=3
  wires:
  Data Store Read/1 -> Control diagnostics/1  "llc1_ts_tbctr"
  Data Store Read2/1 -> Control diagnostics/3  "llc1_burstduty"
  Data Store Read1/1 -> Control diagnostics/2  "llc1_ps"
  Data Store Read3/1 -> Control diagnostics/4  "mode"
  Data Store Read12/1 -> Ref_fbk_fwd/3  "ref_vout"
  Data Store Read4/1 -> Ref_fbk_fwd/1  "ref_iout"
  Data Store Read5/1 -> Ref_fbk_fwd/2  "fbk_iout"
  Data Store Read14/1 -> Multiply/1  "mode"
  Data Store Read6/1 -> Ref_fbk_rev/1  "ref_vbulk"
  Data Store Read8/1 -> Ref_fbk_rev/3  "mode"
  Data Store Read7/1 -> Ref_fbk_rev/2  "fbk_vbulk"
  Data Store Read13/1 -> Ref_fbk_fwd/4  "fbk_vout"
  Multiply/1 -> Ref_fbk_fwd/5
  CP_READY/1 -> control/1(CP_READY)
  AC_OK/1 -> control/2(AC_OK)
  PFC_OK/1 -> control/3(PFC_OK)
  CLLLC_EN/1 -> control/4(CLLLC_EN)
  control/1(PFC_EN) -> Data Type Conversion/1
  control/2(OBC_OK) -> Data Type Conversion1/1
  control/3(CLLLC_OK) -> Data Type Conversion2/1
  Data Type Conversion/1 -> PFC_EN/1
  Data Type Conversion1/1 -> OBC_OK/1
  Data Type Conversion2/1 -> CLLLC_OK/1

== system main/Task_Manager ==
  note: 1mS Tasks
      | For GPIO handler, Protection, Measurement
  note: Idle tasks
  note: System Initialize
  note: Output to simulated plant
  note: 1S Tasks
      | For NTC Mux Handler, Temp Measurement
  note: 20mS Tasks
      | For CAN RX and TX Handler
  tmr_idle : Inport  OutDataTypeStr=single  OutputFunctionCall=on
  signal_digin : Inport  Port=2
  Idle Task1 : idelinklib_common/Idle Task  tasknumbers=[1]  taskpriorities=100017  taskpreempts=[1]  showinput=off  simPriority=0
      settings: SourceProductBaseCode=ME
  Tmr_1mS : Subsystem  Variant=on
  Tmr_1s : Subsystem  Variant=on
  Tmr_20mS : Subsystem  Variant=on
  Variant Sink : VariantSink
  Variant Source2 : VariantSource
      settings: AllowZeroVariantControls=on
  Variant Source4 : VariantSource
      settings: AllowZeroVariantControls=on
  idle : Subsystem
  init : Subsystem  Variant=on
  Out1 : Outport
  signal_digout : Outport  Port=2
  signal_pwm_cllc1 : Outport  Port=3
  wires:
  Variant Source2/1 -> idle/Trigger
  Variant Source4/1 -> idle/1(sim_digin)
  idle/1(sim_digout) -> Variant Sink/1
  Variant Sink/2 -> signal_digout/1
  Idle Task1/1 -> Variant Source2/1
  signal_digin/1 -> Variant Source4/2
  tmr_idle/1 -> Variant Source2/2
  Variant Sink/1 -> Out1/1
  ? -> Variant Source4/1
  [signal_pwm_cllc1] -> signal_pwm_cllc1/1

== system main/interrupt_adca ==
  adca : Inport
  adcb : Inport  Port=2
  function : TriggerPort  TriggerType=function-call  VariantControl=Variant
  Function-Call Generator1 : simulink/Ports & Subsystems/Function-Call Generator  sample_time=-1  numberOfIterations=1  DisallowWideOutput=off
  Function-Call Split1 : FunctionCallSplit  NumOutputPorts=2
  Function-Call Split3 : FunctionCallSplit  NumOutputPorts=2
  Variant Sink : VariantSink
  burst_control : Subsystem  TreatAsAtomicUnit=on
      settings: RTWSystemCode=Inline
  ePWMs : Subsystem
  ePWMs1 : Subsystem  Commented=on
  ePWMs2 : Subsystem  Commented=on
  ePWMs3 : Subsystem  Commented=on
  ePWMs4 : Subsystem  Commented=on
  get_adc : Subsystem  TreatAsAtomicUnit=on
      settings: RTWSystemCode=Inline
  to_simulated_plant : Subsystem  Variant=on
  signal_pwm_cllc1 : Outport
  wires:
  Function-Call Split3/1 -> get_adc/Trigger
  Function-Call Generator1/1 -> Function-Call Split3/1
  adca/1 -> get_adc/1(sim_adca)
  to_simulated_plant/1(signal_pwm_cllc1) -> Variant Sink/1
  Variant Sink/2 -> signal_pwm_cllc1/1
  adcb/1 -> get_adc/2(sim_adcb)
  Function-Call Split1/1 -> burst_control/Trigger
  Function-Call Split3/2 -> Function-Call Split1/1
  Function-Call Split1/2 -> ePWMs/Trigger

== system main/interrupt_canrx ==
  Inport : Inport
  function : TriggerPort  TriggerType=function-call  VariantControl=Variant
  canrx_variant_subsystem : Subsystem  Variant=on  VariantControlMode=label  VariantControl=Choice  LabelModeActiveChoice=sim_en==0
  wires:
  Inport/1 -> canrx_variant_subsystem/1(signal_canrx)

== system main/Control_State_Machine/control/burstLlc1 ==
  note: Note 0
  note: Compensation:
      | P = kP*error
      | I = kI*[error/2 + sum(past_error)]
      | D = kD*[2*error +- 4*sum(past_error)]
  ref : Inport
  input : Inport  Port=2
  burstduty_integ_in : Inport  Port=3  OutDataTypeStr=single
  f : TriggerPort  TriggerType=function-call  VariantControl=(inherit)
      settings: CopyFcn=Stateflow.SLINSF.SimulinkMan.removeBlockPreDeleteFcn  PreDeleteFcn=Stateflow.SLINSF.SimulinkMan.unsafePredeleteFcn
  Constant : Constant  OutDataTypeStr=single
  Constant5 : Constant  Value=0.5  OutDataTypeStr=single
  Data Store Read : DataStoreRead  DataStoreName=burstduty_kp  IndexOptions=Index vector (dialog)  Indices=1  OutputSizes=1
  Data Store Read2 : DataStoreRead  DataStoreName=burstduty_ki  IndexOptions=Index vector (dialog)  Indices=1  OutputSizes=1
  Data Store Read3 : DataStoreRead  DataStoreName=burstduty_integ_max  IndexOptions=Index vector (dialog)  Indices=1  OutputSizes=1
  Data Store Read4 : DataStoreRead  DataStoreName=burstduty_integ_min  IndexOptions=Index vector (dialog)  Indices=1  OutputSizes=1
  Data Type Conversion : DataTypeConversion  OutDataTypeStr=single  SaturateOnIntegerOverflow=off  RndMeth=Floor
  Product1 : Product  Inputs=4
  Product2 : Product
  Saturation Dynamic : simulink/Discontinuities/Saturation Dynamic  OutMin=[]  OutMax=[]  OutDataTypeStr=single  OutputDataTypeScalingMode=single  OutDataType=fixdt(1, 16)  OutScaling=2^-10  DoSatur=off
  Saturation Dynamic1 : simulink/Discontinuities/Saturation Dynamic  OutMin=[]  OutMax=[]  OutDataTypeStr=single  OutputDataTypeScalingMode=single  OutDataType=fixdt(1, 16)  OutScaling=2^-10  DoSatur=off
  Sum2 : Sum  Inputs=2
  Sum3 : Sum  Inputs=|++
  Sum5 : Sum  Inputs=2
  Sum6 : Sum  Inputs=|+-
  burstduty : Scope  NumInputPorts=4
  llc1_burstduty : Outport
  burstduty_integ_out : Outport  Port=2  OutDataTypeStr=single
  wires:
  Constant/1 -> Product1/2
  Data Store Read/1 -> [kp]
  Data Store Read2/1 -> [ki]
  Sum6/1 -> Data Type Conversion/1
  Data Type Conversion/1 -> [error]
  Data Store Read4/1 -> [integ_min]
  Data Store Read3/1 -> [integ_max]
  input/1 -> Sum6/2
  ref/1 -> Sum6/1
  Sum5/1 -> burstduty_integ_out/1
  [integ_max] -> Saturation Dynamic1/1
  [error] -> Product2/1
  [ki] -> Product1/3
  Saturation Dynamic/1 -> Sum3/2
  Saturation Dynamic1/1 -> burstduty/4, llc1_burstduty/1  "llc1_burstduty"
  [integ_min] -> Saturation Dynamic1/3
  [integ_max] -> Saturation Dynamic/1
  Sum3/1 -> burstduty/3, Sum2/1, Sum5/2  "kI_term"
  Product2/1 -> burstduty/2, Sum2/2  "kP_term"
  [integ_min] -> Saturation Dynamic/3
  Constant5/1 -> Product1/4
  Sum2/1 -> Saturation Dynamic1/2
  [error] -> Product1/1
  [kp] -> Product2/2
  Product1/1 -> Sum3/1, Sum5/1
  [error] -> burstduty/1  "error"
  burstduty_integ_in/1 -> [burstduty_integ]
  [burstduty_integ] -> Saturation Dynamic/2

== system main/Control_State_Machine/control/configPowerLimitG2v ==
  note: Note: 0 to 375, and 950
  ref_vbat : Inport
  ref_iout : Inport  Port=2
  f : TriggerPort  TriggerType=function-call  VariantControl=(inherit)
      settings: CopyFcn=Stateflow.SLINSF.SimulinkMan.removeBlockPreDeleteFcn  PreDeleteFcn=Stateflow.SLINSF.SimulinkMan.unsafePredeleteFcn
  If : If  IfExpression=(u1>375)&(u1<950)
  If Action Subsystem : Subsystem  TreatAsAtomicUnit=on
  If Action Subsystem2 : Subsystem  TreatAsAtomicUnit=on
  Merge : Merge
  ref_pout : Outport
  wires:
  If/1 -> If Action Subsystem2/Action
  If/2 -> If Action Subsystem/Action
  [ref_iout] -> If Action Subsystem/2(ref_iout)
  Merge/1 -> ref_pout/1
  [ref_vbat] -> If/1
  [ref_vbat] -> If Action Subsystem/1(ref_vbat)
  If Action Subsystem/1(ref_pout) -> Merge/2
  If Action Subsystem2/1(ref_pout) -> Merge/1
  ref_vbat/1 -> [ref_vbat]
  ref_iout/1 -> [ref_iout]

== system main/Control_State_Machine/control/configSr ==
  dir_v2g : Inport
  f : TriggerPort  TriggerType=function-call  VariantControl=(inherit)
      settings: CopyFcn=Stateflow.SLINSF.SimulinkMan.removeBlockPreDeleteFcn  PreDeleteFcn=Stateflow.SLINSF.SimulinkMan.unsafePredeleteFcn
  configXbarEpwmtrip : Subsystem  Variant=on
  wires:
  dir_v2g/1 -> configXbarEpwmtrip/1(dir_v2g)
